simulink model "wb_spectrometer_16"  (R2012b)
(part 2 of 131)

  posedge1 : Subsystem  AncestorBlock=casper_library_misc/edge_detect  mask(edge_detect){edge=Rising, polarity=Active High, x_in=[0 0.08 0.08 0.16 0.16 0.24 0.24 0.32 0.32 0.4], y_in=[-1 -1  1  1  1  1  1  1  1  1], x_out=[0.6 0.68 0.68 0.76 0.76 0.84 0.84 0.92 0.92 1], y_out=[-1 -1  1  1 -1 -1 -1 -1 -1 -1]}
      mask prompts: edge "Edge Type"; polarity "Output Polarity"; x_in "Input X Positions"; y_in "Input Y Positions"; x_out "Output X Positions"; y_out "Output Y Positions"
      mask help: Output is active for one-cycle after each edge of the specified type (i.e. rising, falling or both).
      mask init: same as wb_spectrometer_16/posedge
      settings: AttributesFormatString=|
      | rising edges
      | active high
      mask Help: Output is active for one-cycle after each edge of the specified type (i.e. rising, falling, or both).  Latency is zero.
      mask TypeOptions edge: Rising | Falling | Both
      mask TypeOptions polarity: Active High | Active Low
      mask Display:
      | plot(x_in_num,0.5+y_in_num*0.2);
      | plot(x_out_num,0.5+y_out_num*0.2);
  posedge10 : Subsystem  AncestorBlock=casper_library_misc/edge_detect  mask(edge_detect){edge=Rising, polarity=Active High, x_in=[0 0.08 0.08 0.16 0.16 0.24 0.24 0.32 0.32 0.4], y_in=[-1 -1  1  1  1  1  1  1  1  1], x_out=[0.6 0.68 0.68 0.76 0.76 0.84 0.84 0.92 0.92 1], y_out=[-1 -1  1  1 -1 -1 -1 -1 -1 -1]}
      mask prompts: edge "Edge Type"; polarity "Output Polarity"; x_in "Input X Positions"; y_in "Input Y Positions"; x_out "Output X Positions"; y_out "Output Y Positions"
      mask help: Output is active for one-cycle after each edge of the specified type (i.e. rising, falling or both).
      mask init: same as wb_spectrometer_16/posedge
      settings: AttributesFormatString=|
      | rising edges
      | active high
      mask Help: Output is active for one-cycle after each edge of the specified type (i.e. rising, falling, or both).  Latency is zero.
      mask TypeOptions edge: Rising | Falling | Both
      mask TypeOptions polarity: Active High | Active Low
      mask Display:
      | plot(x_in_num,0.5+y_in_num*0.2);
      | plot(x_out_num,0.5+y_out_num*0.2);
  posedge11 : Subsystem  AncestorBlock=casper_library_misc/edge_detect  mask(edge_detect){edge=Rising, polarity=Active High, x_in=[0 0.08 0.08 0.16 0.16 0.24 0.24 0.32 0.32 0.4], y_in=[-1 -1  1  1  1  1  1  1  1  1], x_out=[0.6 0.68 0.68 0.76 0.76 0.84 0.84 0.92 0.92 1], y_out=[-1 -1  1  1 -1 -1 -1 -1 -1 -1]}
      mask prompts: edge "Edge Type"; polarity "Output Polarity"; x_in "Input X Positions"; y_in "Input Y Positions"; x_out "Output X Positions"; y_out "Output Y Positions"
      mask help: Output is active for one-cycle after each edge of the specified type (i.e. rising, falling or both).
      mask init: same as wb_spectrometer_16/posedge
      settings: AttributesFormatString=|
      | rising edges
      | active high
      mask Help: Output is active for one-cycle after each edge of the specified type (i.e. rising, falling, or both).  Latency is zero.
      mask TypeOptions edge: Rising | Falling | Both
      mask TypeOptions polarity: Active High | Active Low
      mask Display:
      | plot(x_in_num,0.5+y_in_num*0.2);
      | plot(x_out_num,0.5+y_out_num*0.2);
  posedge12 : Subsystem  AncestorBlock=casper_library_misc/edge_detect  mask(edge_detect){edge=Rising, polarity=Active High, x_in=[0 0.08 0.08 0.16 0.16 0.24 0.24 0.32 0.32 0.4], y_in=[-1 -1  1  1  1  1  1  1  1  1], x_out=[0.6 0.68 0.68 0.76 0.76 0.84 0.84 0.92 0.92 1], y_out=[-1 -1  1  1 -1 -1 -1 -1 -1 -1]}
      mask prompts: edge "Edge Type"; polarity "Output Polarity"; x_in "Input X Positions"; y_in "Input Y Positions"; x_out "Output X Positions"; y_out "Output Y Positions"
      mask help: Output is active for one-cycle after each edge of the specified type (i.e. rising, falling or both).
      mask init: same as wb_spectrometer_16/posedge
      settings: AttributesFormatString=|
      | rising edges
      | active high
      mask Help: Output is active for one-cycle after each edge of the specified type (i.e. rising, falling, or both).  Latency is zero.
      mask TypeOptions edge: Rising | Falling | Both
      mask TypeOptions polarity: Active High | Active Low
      mask Display:
      | plot(x_in_num,0.5+y_in_num*0.2);
      | plot(x_out_num,0.5+y_out_num*0.2);
  posedge13 : Subsystem  AncestorBlock=casper_library_misc/edge_detect  mask(edge_detect){edge=Rising, polarity=Active High, x_in=[0 0.08 0.08 0.16 0.16 0.24 0.24 0.32 0.32 0.4], y_in=[-1 -1  1  1  1  1  1  1  1  1], x_out=[0.6 0.68 0.68 0.76 0.76 0.84 0.84 0.92 0.92 1], y_out=[-1 -1  1  1 -1 -1 -1 -1 -1 -1]}
      mask prompts: edge "Edge Type"; polarity "Output Polarity"; x_in "Input X Positions"; y_in "Input Y Positions"; x_out "Output X Positions"; y_out "Output Y Positions"
      mask help: Output is active for one-cycle after each edge of the specified type (i.e. rising, falling or both).
      mask init: same as wb_spectrometer_16/posedge
      settings: AttributesFormatString=|
      | rising edges
      | active high
      mask Help: Output is active for one-cycle after each edge of the specified type (i.e. rising, falling, or both).  Latency is zero.
      mask TypeOptions edge: Rising | Falling | Both
      mask TypeOptions polarity: Active High | Active Low
      mask Display:
      | plot(x_in_num,0.5+y_in_num*0.2);
      | plot(x_out_num,0.5+y_out_num*0.2);
  posedge14 : Subsystem  AncestorBlock=casper_library_misc/edge_detect  mask(edge_detect){edge=Rising, polarity=Active High, x_in=[0 0.08 0.08 0.16 0.16 0.24 0.24 0.32 0.32 0.4], y_in=[-1 -1  1  1  1  1  1  1  1  1], x_out=[0.6 0.68 0.68 0.76 0.76 0.84 0.84 0.92 0.92 1], y_out=[-1 -1  1  1 -1 -1 -1 -1 -1 -1]}
      mask prompts: edge "Edge Type"; polarity "Output Polarity"; x_in "Input X Positions"; y_in "Input Y Positions"; x_out "Output X Positions"; y_out "Output Y Positions"
      mask help: Output is active for one-cycle after each edge of the specified type (i.e. rising, falling or both).
      mask init: same as wb_spectrometer_16/posedge
      settings: AttributesFormatString=|
      | rising edges
      | active high
      mask Help: Output is active for one-cycle after each edge of the specified type (i.e. rising, falling, or both).  Latency is zero.
      mask TypeOptions edge: Rising | Falling | Both
      mask TypeOptions polarity: Active High | Active Low
      mask Display:
      | plot(x_in_num,0.5+y_in_num*0.2);
      | plot(x_out_num,0.5+y_out_num*0.2);
  posedge15 : Subsystem  AncestorBlock=casper_library_misc/edge_detect  mask(edge_detect){edge=Rising, polarity=Active High, x_in=[0 0.08 0.08 0.16 0.16 0.24 0.24 0.32 0.32 0.4], y_in=[-1 -1  1  1  1  1  1  1  1  1], x_out=[0.6 0.68 0.68 0.76 0.76 0.84 0.84 0.92 0.92 1], y_out=[-1 -1  1  1 -1 -1 -1 -1 -1 -1]}
      mask prompts: edge "Edge Type"; polarity "Output Polarity"; x_in "Input X Positions"; y_in "Input Y Positions"; x_out "Output X Positions"; y_out "Output Y Positions"
      mask help: Output is active for one-cycle after each edge of the specified type (i.e. rising, falling or both).
      mask init: same as wb_spectrometer_16/posedge
      settings: AttributesFormatString=|
      | rising edges
      | active high
      mask Help: Output is active for one-cycle after each edge of the specified type (i.e. rising, falling, or both).  Latency is zero.
      mask TypeOptions edge: Rising | Falling | Both
      mask TypeOptions polarity: Active High | Active Low
      mask Display:
      | plot(x_in_num,0.5+y_in_num*0.2);
      | plot(x_out_num,0.5+y_out_num*0.2);
  posedge16 : Subsystem  AncestorBlock=casper_library_misc/edge_detect  mask(edge_detect){edge=Rising, polarity=Active High, x_in=[0 0.08 0.08 0.16 0.16 0.24 0.24 0.32 0.32 0.4], y_in=[-1 -1  1  1  1  1  1  1  1  1], x_out=[0.6 0.68 0.68 0.76 0.76 0.84 0.84 0.92 0.92 1], y_out=[-1 -1  1  1 -1 -1 -1 -1 -1 -1]}
      mask prompts: edge "Edge Type"; polarity "Output Polarity"; x_in "Input X Positions"; y_in "Input Y Positions"; x_out "Output X Positions"; y_out "Output Y Positions"
      mask help: Output is active for one-cycle after each edge of the specified type (i.e. rising, falling or both).
      mask init: same as wb_spectrometer_16/posedge
      settings: AttributesFormatString=|
      | rising edges
      | active high
      mask Help: Output is active for one-cycle after each edge of the specified type (i.e. rising, falling, or both).  Latency is zero.
      mask TypeOptions edge: Rising | Falling | Both
      mask TypeOptions polarity: Active High | Active Low
      mask Display:
      | plot(x_in_num,0.5+y_in_num*0.2);
      | plot(x_out_num,0.5+y_out_num*0.2);
  posedge17 : Subsystem  AncestorBlock=casper_library_misc/edge_detect  mask(edge_detect){edge=Falling, polarity=Active High, x_in=[0 0.08 0.08 0.16 0.16 0.24 0.24 0.32 0.32 0.4], y_in=[-1 -1  1  1  1  1  1  1  1  1], x_out=[0.6 0.68 0.68 0.76 0.76 0.84 0.84 0.92 0.92 1], y_out=[-1 -1  1  1 -1 -1 -1 -1 -1 -1]}
      mask prompts: edge "Edge Type"; polarity "Output Polarity"; x_in "Input X Positions"; y_in "Input Y Positions"; x_out "Output X Positions"; y_out "Output Y Positions"
      mask help: Output is active for one-cycle after each edge of the specified type (i.e. rising, falling or both).
      mask init: same as wb_spectrometer_16/posedge
      settings: AttributesFormatString=|
      | falling edges
      | active high
      mask Help: Output is active for one-cycle after each edge of the specified type (i.e. rising, falling, or both).  Latency is zero.
      mask TypeOptions edge: Rising | Falling | Both
      mask TypeOptions polarity: Active High | Active Low
      mask Display:
      | plot(x_in_num,0.5+y_in_num*0.2);
      | plot(x_out_num,0.5+y_out_num*0.2);
  posedge18 : Subsystem  AncestorBlock=casper_library_misc/edge_detect  mask(edge_detect){edge=Rising, polarity=Active High, x_in=[0 0.08 0.08 0.16 0.16 0.24 0.24 0.32 0.32 0.4], y_in=[-1 -1  1  1  1  1  1  1  1  1], x_out=[0.6 0.68 0.68 0.76 0.76 0.84 0.84 0.92 0.92 1], y_out=[-1 -1  1  1 -1 -1 -1 -1 -1 -1]}
      mask prompts: edge "Edge Type"; polarity "Output Polarity"; x_in "Input X Positions"; y_in "Input Y Positions"; x_out "Output X Positions"; y_out "Output Y Positions"
      mask help: Output is active for one-cycle after each edge of the specified type (i.e. rising, falling or both).
      mask init: same as wb_spectrometer_16/posedge
      settings: AttributesFormatString=|
      | rising edges
      | active high
      mask Help: Output is active for one-cycle after each edge of the specified type (i.e. rising, falling, or both).  Latency is zero.
      mask TypeOptions edge: Rising | Falling | Both
      mask TypeOptions polarity: Active High | Active Low
      mask Display:
      | plot(x_in_num,0.5+y_in_num*0.2);
      | plot(x_out_num,0.5+y_out_num*0.2);
  posedge19 : Subsystem  AncestorBlock=casper_library_misc/edge_detect  mask(edge_detect){edge=Rising, polarity=Active High, x_in=[0 0.08 0.08 0.16 0.16 0.24 0.24 0.32 0.32 0.4], y_in=[-1 -1  1  1  1  1  1  1  1  1], x_out=[0.6 0.68 0.68 0.76 0.76 0.84 0.84 0.92 0.92 1], y_out=[-1 -1  1  1 -1 -1 -1 -1 -1 -1]}
      mask prompts: edge "Edge Type"; polarity "Output Polarity"; x_in "Input X Positions"; y_in "Input Y Positions"; x_out "Output X Positions"; y_out "Output Y Positions"
      mask help: Output is active for one-cycle after each edge of the specified type (i.e. rising, falling or both).
      mask init: same as wb_spectrometer_16/posedge
      settings: AttributesFormatString=|
      | rising edges
      | active high
      mask Help: Output is active for one-cycle after each edge of the specified type (i.e. rising, falling, or both).  Latency is zero.
      mask TypeOptions edge: Rising | Falling | Both
      mask TypeOptions polarity: Active High | Active Low
      mask Display:
      | plot(x_in_num,0.5+y_in_num*0.2);
      | plot(x_out_num,0.5+y_out_num*0.2);
  posedge2 : Subsystem  AncestorBlock=casper_library_misc/edge_detect  mask(edge_detect){edge=Rising, polarity=Active High, x_in=[0 0.08 0.08 0.16 0.16 0.24 0.24 0.32 0.32 0.4], y_in=[-1 -1  1  1  1  1  1  1  1  1], x_out=[0.6 0.68 0.68 0.76 0.76 0.84 0.84 0.92 0.92 1], y_out=[-1 -1  1  1 -1 -1 -1 -1 -1 -1]}
      mask prompts: edge "Edge Type"; polarity "Output Polarity"; x_in "Input X Positions"; y_in "Input Y Positions"; x_out "Output X Positions"; y_out "Output Y Positions"
      mask help: Output is active for one-cycle after each edge of the specified type (i.e. rising, falling or both).
      mask init: same as wb_spectrometer_16/posedge
      settings: AttributesFormatString=|
      | rising edges
      | active high
      mask Help: Output is active for one-cycle after each edge of the specified type (i.e. rising, falling, or both).  Latency is zero.
      mask TypeOptions edge: Rising | Falling | Both
      mask TypeOptions polarity: Active High | Active Low
      mask Display:
      | plot(x_in_num,0.5+y_in_num*0.2);
      | plot(x_out_num,0.5+y_out_num*0.2);
  posedge3 : Subsystem  AncestorBlock=casper_library_misc/edge_detect  mask(edge_detect){edge=Rising, polarity=Active High, x_in=[0 0.08 0.08 0.16 0.16 0.24 0.24 0.32 0.32 0.4], y_in=[-1 -1  1  1  1  1  1  1  1  1], x_out=[0.6 0.68 0.68 0.76 0.76 0.84 0.84 0.92 0.92 1], y_out=[-1 -1  1  1 -1 -1 -1 -1 -1 -1]}
      mask prompts: edge "Edge Type"; polarity "Output Polarity"; x_in "Input X Positions"; y_in "Input Y Positions"; x_out "Output X Positions"; y_out "Output Y Positions"
      mask help: Output is active for one-cycle after each edge of the specified type (i.e. rising, falling or both).
      mask init: same as wb_spectrometer_16/posedge
      settings: AttributesFormatString=|
      | rising edges
      | active high
      mask Help: Output is active for one-cycle after each edge of the specified type (i.e. rising, falling, or both).  Latency is zero.
      mask TypeOptions edge: Rising | Falling | Both
      mask TypeOptions polarity: Active High | Active Low
      mask Display:
      | plot(x_in_num,0.5+y_in_num*0.2);
      | plot(x_out_num,0.5+y_out_num*0.2);
  posedge4 : Subsystem  AncestorBlock=casper_library_misc/edge_detect  mask(edge_detect){edge=Rising, polarity=Active High, x_in=[0 0.08 0.08 0.16 0.16 0.24 0.24 0.32 0.32 0.4], y_in=[-1 -1  1  1  1  1  1  1  1  1], x_out=[0.6 0.68 0.68 0.76 0.76 0.84 0.84 0.92 0.92 1], y_out=[-1 -1  1  1 -1 -1 -1 -1 -1 -1]}
      mask prompts: edge "Edge Type"; polarity "Output Polarity"; x_in "Input X Positions"; y_in "Input Y Positions"; x_out "Output X Positions"; y_out "Output Y Positions"
      mask help: Output is active for one-cycle after each edge of the specified type (i.e. rising, falling or both).
      mask init: same as wb_spectrometer_16/posedge
      settings: AttributesFormatString=|
      | rising edges
      | active high
      mask Help: Output is active for one-cycle after each edge of the specified type (i.e. rising, falling, or both).  Latency is zero.
      mask TypeOptions edge: Rising | Falling | Both
      mask TypeOptions polarity: Active High | Active Low
      mask Display:
      | plot(x_in_num,0.5+y_in_num*0.2);
      | plot(x_out_num,0.5+y_out_num*0.2);
  posedge5 : Subsystem  AncestorBlock=casper_library_misc/edge_detect  mask(edge_detect){edge=Rising, polarity=Active High, x_in=[0 0.08 0.08 0.16 0.16 0.24 0.24 0.32 0.32 0.4], y_in=[-1 -1  1  1  1  1  1  1  1  1], x_out=[0.6 0.68 0.68 0.76 0.76 0.84 0.84 0.92 0.92 1], y_out=[-1 -1  1  1 -1 -1 -1 -1 -1 -1]}
      mask prompts: edge "Edge Type"; polarity "Output Polarity"; x_in "Input X Positions"; y_in "Input Y Positions"; x_out "Output X Positions"; y_out "Output Y Positions"
      mask help: Output is active for one-cycle after each edge of the specified type (i.e. rising, falling or both).
      mask init: same as wb_spectrometer_16/posedge
      settings: AttributesFormatString=|
      | rising edges
      | active high
      mask Help: Output is active for one-cycle after each edge of the specified type (i.e. rising, falling, or both).  Latency is zero.
      mask TypeOptions edge: Rising | Falling | Both
      mask TypeOptions polarity: Active High | Active Low
      mask Display:
      | plot(x_in_num,0.5+y_in_num*0.2);
      | plot(x_out_num,0.5+y_out_num*0.2);
  posedge6 : Subsystem  AncestorBlock=casper_library_misc/edge_detect  mask(edge_detect){edge=Rising, polarity=Active High, x_in=[0 0.08 0.08 0.16 0.16 0.24 0.24 0.32 0.32 0.4], y_in=[-1 -1  1  1  1  1  1  1  1  1], x_out=[0.6 0.68 0.68 0.76 0.76 0.84 0.84 0.92 0.92 1], y_out=[-1 -1  1  1 -1 -1 -1 -1 -1 -1]}
      mask prompts: edge "Edge Type"; polarity "Output Polarity"; x_in "Input X Positions"; y_in "Input Y Positions"; x_out "Output X Positions"; y_out "Output Y Positions"
      mask help: Output is active for one-cycle after each edge of the specified type (i.e. rising, falling or both).
      mask init: same as wb_spectrometer_16/posedge
      settings: AttributesFormatString=|
      | rising edges
      | active high
      mask Help: Output is active for one-cycle after each edge of the specified type (i.e. rising, falling, or both).  Latency is zero.
      mask TypeOptions edge: Rising | Falling | Both
      mask TypeOptions polarity: Active High | Active Low
      mask Display:
      | plot(x_in_num,0.5+y_in_num*0.2);
      | plot(x_out_num,0.5+y_out_num*0.2);
  posedge8 : Subsystem  AncestorBlock=casper_library_misc/edge_detect  mask(edge_detect){edge=Rising, polarity=Active High, x_in=[0 0.08 0.08 0.16 0.16 0.24 0.24 0.32 0.32 0.4], y_in=[-1 -1  1  1  1  1  1  1  1  1], x_out=[0.6 0.68 0.68 0.76 0.76 0.84 0.84 0.92 0.92 1], y_out=[-1 -1  1  1 -1 -1 -1 -1 -1 -1]}
      mask prompts: edge "Edge Type"; polarity "Output Polarity"; x_in "Input X Positions"; y_in "Input Y Positions"; x_out "Output X Positions"; y_out "Output Y Positions"
      mask help: Output is active for one-cycle after each edge of the specified type (i.e. rising, falling or both).
      mask init: same as wb_spectrometer_16/posedge
      settings: AttributesFormatString=|
      | rising edges
      | active high
      mask Help: Output is active for one-cycle after each edge of the specified type (i.e. rising, falling, or both).  Latency is zero.
      mask TypeOptions edge: Rising | Falling | Both
      mask TypeOptions polarity: Active High | Active Low
      mask Display:
      | plot(x_in_num,0.5+y_in_num*0.2);
      | plot(x_out_num,0.5+y_out_num*0.2);
  posedge9 : Subsystem  AncestorBlock=casper_library_misc/edge_detect  mask(edge_detect){edge=Rising, polarity=Active High, x_in=[0 0.08 0.08 0.16 0.16 0.24 0.24 0.32 0.32 0.4], y_in=[-1 -1  1  1  1  1  1  1  1  1], x_out=[0.6 0.68 0.68 0.76 0.76 0.84 0.84 0.92 0.92 1], y_out=[-1 -1  1  1 -1 -1 -1 -1 -1 -1]}
      mask prompts: edge "Edge Type"; polarity "Output Polarity"; x_in "Input X Positions"; y_in "Input Y Positions"; x_out "Output X Positions"; y_out "Output Y Positions"
      mask help: Output is active for one-cycle after each edge of the specified type (i.e. rising, falling or both).
      mask init: same as wb_spectrometer_16/posedge
      settings: AttributesFormatString=|
      | rising edges
      | active high
      mask Help: Output is active for one-cycle after each edge of the specified type (i.e. rising, falling, or both).  Latency is zero.
      mask TypeOptions edge: Rising | Falling | Both
      mask TypeOptions polarity: Active High | Active Low
      mask Display:
      | plot(x_in_num,0.5+y_in_num*0.2);
      | plot(x_out_num,0.5+y_out_num*0.2);
  pps_ : xbsIndex_r4/Gateway Out  inherit_from_input=off  hdl_port=on  timing_constraint=None  locs_specified=off  LOCs={}  UseAsDAC=off  DACChannel='1'  block_type=gatewayout
  pps_cnt : Subsystem  Tag=xps:sw_reg  AncestorBlock=xps_library/software register  mask(swreg){mode=one value, io_dir=To Processor, io_delay=0, sample_period=1, names=reg, bitwidths=32, arith_types=0, bin_pts=0, sim_port=on, show_format=off}
      mask prompts: io_dir "I/O direction"; io_delay "I/O delay"; sample_period "Sample period"; names "Name:"; bitwidths "Bitwidth:"; arith_types "Type (ufix=0, fix=1, bool=2):"; bin_pts "Binary pt:"; sim_port "Provide sim input/output?"; show_format "Print format string?"
      mask init:
      | swreg_init(gcb)
      settings: AttributesFormatString=1output
      mask TypeOptions mode: one value | fields of equal size | fields of arbitrary size
      mask Callback mode: swreg_cb(gcb);
      mask TypeOptions io_dir: To Processor | From Processor
      mask Callback io_dir:
      | mask_enables = get_param(gcb, 'MaskEnables');
      | mask_names = get_param(gcb, 'MaskNames');
      | if strcmp(get_param(gcb, 'io_dir'), 'To Processor'),
      |     mask_enables{ismember(mask_names, 'sample_period')} = 'off';
      | else
      |     mask_enables{ismember(mask_names, 'sample_period')} = 'on';
      | end
      | set_param(gcb, 'MaskEnables', mask_enables);
      mask Callback bitwidths: swreg_maskcheck(gcb);
      mask Callback arith_types: [numios, ~, ~, ~, current_types] = swreg_maskcheck(gcb);
      mask Callback bin_pts: swreg_maskcheck(gcb);
  queue_empty : Subsystem  Tag=xps:sw_reg  AncestorBlock=xps_library/software register  mask(swreg){mode=one value, io_dir=To Processor, io_delay=0, sample_period=1, names=reg, bitwidths=1, arith_types=2, bin_pts=0, sim_port=on, show_format=off}
      mask prompts: io_dir "I/O direction"; io_delay "I/O delay"; sample_period "Sample period"; names "Name:"; bitwidths "Bitwidth:"; arith_types "Type (ufix=0, fix=1, bool=2):"; bin_pts "Binary pt:"; sim_port "Provide sim input/output?"; show_format "Print format string?"
      mask init:
      | swreg_init(gcb)
      settings: AttributesFormatString=1output
      mask TypeOptions mode: one value | fields of equal size | fields of arbitrary size
      mask Callback mode: swreg_cb(gcb);
      mask TypeOptions io_dir: To Processor | From Processor
      mask Callback io_dir:
      | mask_enables = get_param(gcb, 'MaskEnables');
      | mask_names = get_param(gcb, 'MaskNames');
      | if strcmp(get_param(gcb, 'io_dir'), 'To Processor'),
      |     mask_enables{ismember(mask_names, 'sample_period')} = 'off';
      | else
      |     mask_enables{ismember(mask_names, 'sample_period')} = 'on';
      | end
      | set_param(gcb, 'MaskEnables', mask_enables);
      mask Callback bitwidths: swreg_maskcheck(gcb);
      mask Callback arith_types: [numios, ~, ~, ~, current_types] = swreg_maskcheck(gcb);
      mask Callback bin_pts: swreg_maskcheck(gcb);
  queue_perc_full : Subsystem  Tag=xps:sw_reg  AncestorBlock=xps_library/software register  mask(swreg){mode=one value, io_dir=To Processor, io_delay=0, sample_period=1, names=reg, bitwidths=8, arith_types=0, bin_pts=8, sim_port=on, show_format=off}
      mask prompts: io_dir "I/O direction"; io_delay "I/O delay"; sample_period "Sample period"; names "Name:"; bitwidths "Bitwidth:"; arith_types "Type (ufix=0, fix=1, bool=2):"; bin_pts "Binary pt:"; sim_port "Provide sim input/output?"; show_format "Print format string?"
      mask init:
      | swreg_init(gcb)
      settings: AttributesFormatString=1output
      mask TypeOptions mode: one value | fields of equal size | fields of arbitrary size
      mask Callback mode: swreg_cb(gcb);
      mask TypeOptions io_dir: To Processor | From Processor
      mask Callback io_dir:
      | mask_enables = get_param(gcb, 'MaskEnables');
      | mask_names = get_param(gcb, 'MaskNames');
      | if strcmp(get_param(gcb, 'io_dir'), 'To Processor'),
      |     mask_enables{ismember(mask_names, 'sample_period')} = 'off';
      | else
      |     mask_enables{ismember(mask_names, 'sample_period')} = 'on';
      | end
      | set_param(gcb, 'MaskEnables', mask_enables);
      mask Callback bitwidths: swreg_maskcheck(gcb);
      mask Callback arith_types: [numios, ~, ~, ~, current_types] = swreg_maskcheck(gcb);
      mask Callback bin_pts: swreg_maskcheck(gcb);
  roach_gpio_a_enable_not : xps_library/gpio  Tag=xps:gpio  io_group=ROACH:gpioa_oe_n  io_dir=out  arith_type=Boolean  bitwidth=1  bin_pt=0  bit_index=0  sample_period=1  use_single_ended=off  use_ddr=off  reg_iob=off  reg_clk_phase=0  termination=None
      link override convert: arith_type=Boolean  n_bits=1  bin_pt=0
  roach_gpio_b_enable_not : xps_library/gpio  Tag=xps:gpio  io_group=ROACH:gpiob_oe_n  io_dir=out  arith_type=Boolean  bitwidth=1  bin_pt=0  bit_index=0  sample_period=1  use_single_ended=off  use_ddr=off  reg_iob=off  reg_clk_phase=0  termination=None
      link override convert: arith_type=Boolean  n_bits=1  bin_pt=0
  roach_led0 : xps_library/gpio  Tag=xps:gpio  io_group=ROACH:gpiob  io_dir=out  arith_type=Boolean  bitwidth=1  bin_pt=0  bit_index=0  sample_period=1  use_single_ended=off  use_ddr=off  reg_iob=off  reg_clk_phase=0  termination=None
      link override convert: arith_type=Boolean  n_bits=1  bin_pt=0
  roach_led1 : xps_library/gpio  Tag=xps:gpio  io_group=ROACH:gpiob  io_dir=out  arith_type=Boolean  bitwidth=1  bin_pt=0  bit_index=1  sample_period=1  use_single_ended=off  use_ddr=off  reg_iob=off  reg_clk_phase=0  termination=None
      link override convert: arith_type=Boolean  n_bits=1  bin_pt=0
  roach_led2 : xps_library/gpio  Tag=xps:gpio  io_group=ROACH:gpiob  io_dir=out  arith_type=Boolean  bitwidth=1  bin_pt=0  bit_index=2  sample_period=1  use_single_ended=off  use_ddr=off  reg_iob=off  reg_clk_phase=0  termination=None
      link override convert: arith_type=Boolean  n_bits=1  bin_pt=0
  roach_led3 : xps_library/gpio  Tag=xps:gpio  io_group=ROACH:gpiob  io_dir=out  arith_type=Boolean  bitwidth=1  bin_pt=0  bit_index=3  sample_period=1  use_single_ended=off  use_ddr=off  reg_iob=off  reg_clk_phase=0  termination=None
      link override convert: arith_type=Boolean  n_bits=1  bin_pt=0
  roach_led4 : xps_library/gpio  Tag=xps:gpio  io_group=ROACH:gpiob  io_dir=out  arith_type=Boolean  bitwidth=1  bin_pt=0  bit_index=4  sample_period=1  use_single_ended=off  use_ddr=off  reg_iob=off  reg_clk_phase=0  termination=None
      link override convert: arith_type=Boolean  n_bits=1  bin_pt=0
  roach_led5 : xps_library/gpio  Tag=xps:gpio  io_group=ROACH:gpiob  io_dir=out  arith_type=Boolean  bitwidth=1  bin_pt=0  bit_index=5  sample_period=1  use_single_ended=off  use_ddr=off  reg_iob=off  reg_clk_phase=0  termination=None
      link override convert: arith_type=Boolean  n_bits=1  bin_pt=0
  roach_led6 : xps_library/gpio  Tag=xps:gpio  io_group=ROACH:gpiob  io_dir=out  arith_type=Boolean  bitwidth=1  bin_pt=0  bit_index=6  sample_period=1  use_single_ended=off  use_ddr=off  reg_iob=off  reg_clk_phase=0  termination=None
      link override convert: arith_type=Boolean  n_bits=1  bin_pt=0
  roach_led7 : xps_library/gpio  Tag=xps:gpio  io_group=ROACH:gpiob  io_dir=out  arith_type=Boolean  bitwidth=1  bin_pt=0  bit_index=7  sample_period=1  use_single_ended=off  use_ddr=off  reg_iob=off  reg_clk_phase=0  termination=None
      link override convert: arith_type=Boolean  n_bits=1  bin_pt=0
  roach_sma_j10 : xps_library/gpio  Tag=xps:gpio  io_group=ROACH:gpioa  io_dir=out  arith_type=Boolean  bitwidth=1  bin_pt=0  bit_index=4  sample_period=1  use_single_ended=off  use_ddr=off  reg_iob=off  reg_clk_phase=0  termination=None
      link override convert: arith_type=Boolean  n_bits=1  bin_pt=0
  rtc_ : xbsIndex_r4/Gateway Out  inherit_from_input=off  hdl_port=on  timing_constraint=None  locs_specified=off  LOCs={}  UseAsDAC=off  DACChannel='1'  block_type=gatewayout
  sampling_frequency_mhz : Subsystem  Tag=xps:sw_reg  AncestorBlock=xps_library/software register  mask(swreg){mode=one value, io_dir=To Processor, io_delay=0, sample_period=1, names=reg, bitwidths=32, arith_types=0, bin_pts=0, sim_port=on, show_format=off}
      mask prompts: io_dir "I/O direction"; io_delay "I/O delay"; sample_period "Sample period"; names "Name:"; bitwidths "Bitwidth:"; arith_types "Type (ufix=0, fix=1, bool=2):"; bin_pts "Binary pt:"; sim_port "Provide sim input/output?"; show_format "Print format string?"
      mask init:
      | swreg_init(gcb)
      settings: AttributesFormatString=1output
      mask TypeOptions mode: one value | fields of equal size | fields of arbitrary size
      mask Callback mode: swreg_cb(gcb);
      mask TypeOptions io_dir: To Processor | From Processor
      mask Callback io_dir:
      | mask_enables = get_param(gcb, 'MaskEnables');
      | mask_names = get_param(gcb, 'MaskNames');
      | if strcmp(get_param(gcb, 'io_dir'), 'To Processor'),
      |     mask_enables{ismember(mask_names, 'sample_period')} = 'off';
      | else
      |     mask_enables{ismember(mask_names, 'sample_period')} = 'on';
      | end
      | set_param(gcb, 'MaskEnables', mask_enables);
      mask Callback bitwidths: swreg_maskcheck(gcb);
      mask Callback arith_types: [numios, ~, ~, ~, current_types] = swreg_maskcheck(gcb);
      mask Callback bin_pts: swreg_maskcheck(gcb);
  simple_bram_vacc_i_even : Subsystem  AncestorBlock=casper_library_accumulators/simple_bram_vacc  mask(simple_bram_vacc){vec_len=512, arith_type=Signed, n_bits=32, bin_pt=0}
      mask prompts: vec_len "Vector length:"; arith_type "Output type:"; n_bits "Bit width (output):"; bin_pt "Binary point (output):"
      mask help: This simple vector accumulator is based on a shift register. It outputs its previous accumulated vector after a new_acc pulse is received.
      mask init:
      | simple_bram_vacc_init(gcb, ...
      |     'vec_len', vec_len, ...
      |     'arith_type', arith_type, ...
      |     'n_bits', n_bits, ...
      |     'bin_pt', bin_pt);
      mask TypeOptions arith_type: Signed | Unsigned
  simple_bram_vacc_i_odd : Subsystem  AncestorBlock=casper_library_accumulators/simple_bram_vacc  mask(simple_bram_vacc){vec_len=512, arith_type=Signed, n_bits=32, bin_pt=0}
      mask prompts: vec_len "Vector length:"; arith_type "Output type:"; n_bits "Bit width (output):"; bin_pt "Binary point (output):"
      mask help: This simple vector accumulator is based on a shift register. It outputs its previous accumulated vector after a new_acc pulse is received.
      mask init:
      | simple_bram_vacc_init(gcb, ...
      |     'vec_len', vec_len, ...
      |     'arith_type', arith_type, ...
      |     'n_bits', n_bits, ...
      |     'bin_pt', bin_pt);
      mask TypeOptions arith_type: Signed | Unsigned
  simple_bram_vacc_q_even : Subsystem  AncestorBlock=casper_library_accumulators/simple_bram_vacc  mask(simple_bram_vacc){vec_len=512, arith_type=Signed, n_bits=32, bin_pt=0}
      mask prompts: vec_len "Vector length:"; arith_type "Output type:"; n_bits "Bit width (output):"; bin_pt "Binary point (output):"
      mask help: This simple vector accumulator is based on a shift register. It outputs its previous accumulated vector after a new_acc pulse is received.
      mask init:
      | simple_bram_vacc_init(gcb, ...
      |     'vec_len', vec_len, ...
      |     'arith_type', arith_type, ...
      |     'n_bits', n_bits, ...
      |     'bin_pt', bin_pt);
      mask TypeOptions arith_type: Signed | Unsigned
  simple_bram_vacc_q_odd : Subsystem  AncestorBlock=casper_library_accumulators/simple_bram_vacc  mask(simple_bram_vacc){vec_len=512, arith_type=Signed, n_bits=32, bin_pt=0}
      mask prompts: vec_len "Vector length:"; arith_type "Output type:"; n_bits "Bit width (output):"; bin_pt "Binary point (output):"
      mask help: This simple vector accumulator is based on a shift register. It outputs its previous accumulated vector after a new_acc pulse is received.
      mask init:
      | simple_bram_vacc_init(gcb, ...
      |     'vec_len', vec_len, ...
      |     'arith_type', arith_type, ...
      |     'n_bits', n_bits, ...
      |     'bin_pt', bin_pt);
      mask TypeOptions arith_type: Signed | Unsigned
  simple_bram_vacc_u_even : Subsystem  AncestorBlock=casper_library_accumulators/simple_bram_vacc  mask(simple_bram_vacc){vec_len=512, arith_type=Signed, n_bits=32, bin_pt=0}
      mask prompts: vec_len "Vector length:"; arith_type "Output type:"; n_bits "Bit width (output):"; bin_pt "Binary point (output):"
      mask help: This simple vector accumulator is based on a shift register. It outputs its previous accumulated vector after a new_acc pulse is received.
      mask init:
      | simple_bram_vacc_init(gcb, ...
      |     'vec_len', vec_len, ...
      |     'arith_type', arith_type, ...
      |     'n_bits', n_bits, ...
      |     'bin_pt', bin_pt);
      mask TypeOptions arith_type: Signed | Unsigned
  simple_bram_vacc_u_odd : Subsystem  AncestorBlock=casper_library_accumulators/simple_bram_vacc  mask(simple_bram_vacc){vec_len=512, arith_type=Signed, n_bits=32, bin_pt=0}
      mask prompts: vec_len "Vector length:"; arith_type "Output type:"; n_bits "Bit width (output):"; bin_pt "Binary point (output):"
      mask help: This simple vector accumulator is based on a shift register. It outputs its previous accumulated vector after a new_acc pulse is received.
      mask init:
      | simple_bram_vacc_init(gcb, ...
      |     'vec_len', vec_len, ...
      |     'arith_type', arith_type, ...
      |     'n_bits', n_bits, ...
      |     'bin_pt', bin_pt);
      mask TypeOptions arith_type: Signed | Unsigned
  simple_bram_vacc_v_even : Subsystem  AncestorBlock=casper_library_accumulators/simple_bram_vacc  mask(simple_bram_vacc){vec_len=512, arith_type=Signed, n_bits=32, bin_pt=0}
      mask prompts: vec_len "Vector length:"; arith_type "Output type:"; n_bits "Bit width (output):"; bin_pt "Binary point (output):"
      mask help: This simple vector accumulator is based on a shift register. It outputs its previous accumulated vector after a new_acc pulse is received.
      mask init:
      | simple_bram_vacc_init(gcb, ...
      |     'vec_len', vec_len, ...
      |     'arith_type', arith_type, ...
      |     'n_bits', n_bits, ...
      |     'bin_pt', bin_pt);
      mask TypeOptions arith_type: Signed | Unsigned
  simple_bram_vacc_v_odd : Subsystem  AncestorBlock=casper_library_accumulators/simple_bram_vacc  mask(simple_bram_vacc){vec_len=512, arith_type=Signed, n_bits=32, bin_pt=0}
      mask prompts: vec_len "Vector length:"; arith_type "Output type:"; n_bits "Bit width (output):"; bin_pt "Binary point (output):"
      mask help: This simple vector accumulator is based on a shift register. It outputs its previous accumulated vector after a new_acc pulse is received.
      mask init:
      | simple_bram_vacc_init(gcb, ...
      |     'vec_len', vec_len, ...
      |     'arith_type', arith_type, ...
      |     'n_bits', n_bits, ...
      |     'bin_pt', bin_pt);
      mask TypeOptions arith_type: Signed | Unsigned
  stokes_enable : Subsystem  Tag=xps:sw_reg  AncestorBlock=xps_library/software register  mask(swreg){mode=one value, io_dir=From Processor, io_delay=0, sample_period=1, names=reg, bitwidths=32, arith_types=0, bin_pts=0, sim_port=on, show_format=off}
      mask prompts: io_dir "I/O direction"; io_delay "I/O delay"; sample_period "Sample period"; names "Name:"; bitwidths "Bitwidth:"; arith_types "Type (ufix=0, fix=1, bool=2):"; bin_pts "Binary pt:"; sim_port "Provide sim input/output?"; show_format "Print format string?"
      mask init:
      | swreg_init(gcb)
      settings: AttributesFormatString=1input
      mask TypeOptions mode: one value | fields of equal size | fields of arbitrary size
      mask Callback mode: swreg_cb(gcb);
      mask TypeOptions io_dir: To Processor | From Processor
      mask Callback io_dir:
      | mask_enables = get_param(gcb, 'MaskEnables');
      | mask_names = get_param(gcb, 'MaskNames');
      | if strcmp(get_param(gcb, 'io_dir'), 'To Processor'),
      |     mask_enables{ismember(mask_names, 'sample_period')} = 'off';
      | else
      |     mask_enables{ismember(mask_names, 'sample_period')} = 'on';
      | end
      | set_param(gcb, 'MaskEnables', mask_enables);
      mask Callback bitwidths:
      | swreg_maskcheck(gcb);
      | % blk = gcb;
      | % mode = get_param(blk, 'mode');
      | % current_widths = eval(get_param(blk, 'bitwidths'));
      | % if (strcmp(mode, 'one value') || strcmp(mode, 'fields of equal size')) && (length(current_widths) > 1),
      | %     error('Only one width may be specified for this mode.');
      | % elseif strcmp(mode, 'fields of arbitrary size')
      | %     current_names = textscan(strtrim(strrep(strrep(get_param(blk, 'names'), ']', ''), '[', '')), '%s');
      | %     current_names = current_names{1};
      | %     numios = length(current_names);
      | %     if length(current_widths) ~= numios,
      | %         error('%d field names specified, but %d widths?', numios, length(current_widths));
      | %     end
      | % end
      | % total_width = 0;
      | % for ctr = 1 : length(current_widths),
      | %     total_width = total_width + current_widths(ctr);
      | % end
      | % if total_width > 32,
      | %     error('Total width must be 32 or less, set to %d.', total_width);
      | % end
      mask Callback arith_types:
      | [numios, ~, ~, ~, current_types] = swreg_maskcheck(gcb);
      | % blk = gcb;
      | % mode = get_param(blk, 'mode');
      | % current_types = eval(get_param(blk, 'arith_types'));
      | % numios = length(current_types);
      | % if (strcmp(mode, 'one value') || strcmp(mode, 'fields of equal size')) && (length(current_types) > 1),
      | %     error('Only one type may be specified for this mode.');
      | % elseif strcmp(mode, 'fields of arbitrary size')
      | %     current_names = textscan(strtrim(strrep(strrep(get_param(blk, 'names'), ']', ''), '[', '')), '%s');
      | %     current_names = current_names{1};
      | %     numios = length(current_names);
      | %     if length(current_types) ~= numios,
      | %         error('%d field names specified, but %d types?', numios, length(current_types));
      | %     end
      | % end
      | problem = 0;
      | for ctr = 1 : numios,
      |     t = current_types(ctr);
      |     if (t < 0) || (t > 2),
      |         problem = t;
      |         ctr = numios + 1;
      |     end
      | end
      | if problem ~= 0,
      |     error('Type cannot be %i, must be 0, 1 or 2.', problem);
      | end
      mask Callback bin_pts:
      | swreg_maskcheck(gcb);
      | % blk = gcb;
      | % mode = get_param(blk, 'mode');
      | % current_bins = eval(get_param(blk, 'bin_pts'));
      | % if (strcmp(mode, 'one value') || strcmp(mode, 'fields of equal size')) && (length(current_bins) > 1),
      | %     error('Only one binary pt may be specified for this mode.');
      | % elseif strcmp(mode, 'fields of arbitrary size')
      | %     current_names = textscan(strtrim(strrep(strrep(get_param(blk, 'names'), ']', ''), '[', '')), '%s');
      | %     current_names = current_names{1};
      | %     numios = length(current_names);
      | %     if length(current_bins) ~= numios,
      | %         error('%d field names specified, but %d binary pts?', numios, length(current_bins));
      | %     end
      | % end
  stokes_even : Subsystem
  stokes_odd : Subsystem
  sub_frame_cnt : xbsIndex_r4/Counter  cnt_type=Free Running  cnt_to=Inf  operation=Up  start_count=0  cnt_by_val=1  arith_type=Unsigned  n_bits=8  bin_pt=0  load_pin=off  rst=on  en=on  explicit_period=on  period=1  dbl_ovrd=off  use_behavioral_HDL=off  implementation=Fabric  block_type=counter
      settings: block_version=11.4
  sync_next_pps : Subsystem  Tag=xps:sw_reg  AncestorBlock=xps_library/software register  DataTypeOverride=Double  DataTypeOverrideAppliesTo=Fixed-point  MinMaxOverflowLogging=ForceOff  mask(swreg){mode=one value, io_dir=From Processor, io_delay=0, sample_period=1, names=reg, bitwidths=32, arith_types=0, bin_pts=[0], sim_port=on, show_format=off}
      mask prompts: io_dir "I/O direction"; io_delay "I/O delay"; sample_period "Sample period"; names "Name:"; bitwidths "Bitwidth:"; arith_types "Type (ufix=0, fix=1, bool=2):"; bin_pts "Binary pt:"; sim_port "Provide sim input/output?"; show_format "Print format string?"
      mask init:
      | swreg_init(gcb)
      settings: AttributesFormatString=1input
      mask TypeOptions mode: one value | fields of equal size | fields of arbitrary size
      mask Callback mode: swreg_cb(gcb);
      mask TypeOptions io_dir: To Processor | From Processor
      mask Callback io_dir:
      | mask_enables = get_param(gcb, 'MaskEnables');
      | mask_names = get_param(gcb, 'MaskNames');
      | if strcmp(get_param(gcb, 'io_dir'), 'To Processor'),
      |     mask_enables{ismember(mask_names, 'sample_period')} = 'off';
      | else
      |     mask_enables{ismember(mask_names, 'sample_period')} = 'on';
      | end
      | set_param(gcb, 'MaskEnables', mask_enables);
      mask Callback bitwidths:
      | swreg_maskcheck(gcb);
      | % blk = gcb;
      | % mode = get_param(blk, 'mode');
      | % current_widths = eval(get_param(blk, 'bitwidths'));
      | % if (strcmp(mode, 'one value') || strcmp(mode, 'fields of equal size')) && (length(current_widths) > 1),
      | %     error('Only one width may be specified for this mode.');
      | % elseif strcmp(mode, 'fields of arbitrary size')
      | %     current_names = textscan(strtrim(strrep(strrep(get_param(blk, 'names'), ']', ''), '[', '')), '%s');
      | %     current_names = current_names{1};
      | %     numios = length(current_names);
      | %     if length(current_widths) ~= numios,
      | %         error('%d field names specified, but %d widths?', numios, length(current_widths));
      | %     end
      | % end
      | % total_width = 0;
      | % for ctr = 1 : length(current_widths),
      | %     total_width = total_width + current_widths(ctr);
      | % end
      | % if total_width > 32,
      | %     error('Total width must be 32 or less, set to %d.', total_width);
      | % end
      mask Callback arith_types:
      | [numios, ~, ~, ~, current_types] = swreg_maskcheck(gcb);
      | % blk = gcb;
      | % mode = get_param(blk, 'mode');
      | % current_types = eval(get_param(blk, 'arith_types'));
      | % numios = length(current_types);
      | % if (strcmp(mode, 'one value') || strcmp(mode, 'fields of equal size')) && (length(current_types) > 1),
      | %     error('Only one type may be specified for this mode.');
      | % elseif strcmp(mode, 'fields of arbitrary size')
      | %     current_names = textscan(strtrim(strrep(strrep(get_param(blk, 'names'), ']', ''), '[', '')), '%s');
      | %     current_names = current_names{1};
      | %     numios = length(current_names);
      | %     if length(current_types) ~= numios,
      | %         error('%d field names specified, but %d types?', numios, length(current_types));
      | %     end
      | % end
      | problem = 0;
      | for ctr = 1 : numios,
      |     t = current_types(ctr);
      |     if (t < 0) || (t > 2),
      |         problem = t;
      |         ctr = numios + 1;
      |     end
      | end
      | if problem ~= 0,
      |     error('Type cannot be %i, must be 0, 1 or 2.', problem);
      | end
      mask Callback bin_pts:
      | swreg_maskcheck(gcb);
      | % blk = gcb;
      | % mode = get_param(blk, 'mode');
      | % current_bins = eval(get_param(blk, 'bin_pts'));
      | % if (strcmp(mode, 'one value') || strcmp(mode, 'fields of equal size')) && (length(current_bins) > 1),
      | %     error('Only one binary pt may be specified for this mode.');
      | % elseif strcmp(mode, 'fields of arbitrary size')
      | %     current_names = textscan(strtrim(strrep(strrep(get_param(blk, 'names'), ']', ''), '[', '')), '%s');
      | %     current_names = current_names{1};
      | %     numios = length(current_names);
      | %     if length(current_bins) ~= numios,
      | %         error('%d field names specified, but %d binary pts?', numios, length(current_bins));
      | %     end
      | % end
  sync_pulse_ : xbsIndex_r4/Gateway Out  inherit_from_input=off  hdl_port=on  timing_constraint=None  locs_specified=off  LOCs={}  UseAsDAC=off  DACChannel='1'  block_type=gatewayout
  tgbe0 : Subsystem  Tag=xps:tengbe_v2  AncestorBlock=xps_library/ten_Gbe_v2  mask(ten_GbE_v2){flavour=cx4, slot=1, port_r1=2, port_r2_cx4=0, port_r2_sfpp=0, rx_dist_ram=on, large_frames=off, show_param=on, pre_emph_r2=0.74, pre_emph=3, post_emph_r2=0.18, rxeqmix_r2=7, swing_r2=940, swing=800, fab_en=on, fab_mac=hex2dec('123456780000'), fab_ip=10*(2^24) + 0*(2^16) + 0*(2^8) + 2*(2^0), fab_udp=60001, fab_gate=1, cpu_rx_en=on, cpu_tx_en=on, ttl=hex2dec('FF'), promisc_mode=off, debug_ctr_width=16, txctr=on, txerrctr=off, txerrctr_len=4224, txofctr=on, txfullctr=off, txvldctr=on, txsnaplen=8192, rxctr=off, rxerrctr=off, rxerrctr_len=100, rxofctr=off, rxbadctr=off, rxvldctr=off, rxeofctr=off, rxsnaplen=0 - no snap}
      mask prompts: flavour "Mezzanine card flavour"; slot "Card slot"; port_r1 "Port"; port_r2_cx4 "Port"; port_r2_sfpp "Port"; rx_dist_ram "Shallow RX Fifo (Beware overruns!)"; large_frames "Enable Large TX Frames (8k+512)"; show_param "---------------------- Show Implementation Parameters -----------------------------------------------------------------------------------"; pre_emph_r2 "Pre-emphasis (dB)"; pre_emph "Pre-emphasis"; post_emph_r2 "Post-emphasis (dB)"; rxeqmix_r2 "Receive equalisation"; swing_r2 "Driver Swing Control (mVppd)"; swing "Differential swing"; fab_en "Enable fabric on startup"; fab_mac "Fabric MAC Address"; fab_ip "Fabric IP Address"; fab_udp "Fabric UDP Port"; fab_gate "Fabric Gateway"; cpu_rx_en "Enable CPU RX"; cpu_tx_en "Enable CPU TX"; promisc_mode "Promiscuous mode"; debug_ctr_width "Debug counter width"; txctr "TX - core_txctr"; txerrctr "TX packet length error - core_txerrctr"; txerrctr_len "-- expected TX packet length"; txofctr "TX overflow - core_txofctr"; txfullctr "TX full - core_txfullctr"; txvldctr "TX valid cycle - core_txvldctr"; txsnaplen "TX snapshot length"; rxctr "RX - core_rxctr"; rxerrctr "RX packet length error - core_rxerrctr"; rxerrctr_len "-- expected RX packet length"; rxofctr "RX overflow - core_rxofctr"; rxbadctr "RX bad - core_rxbadctr"; rxvldctr "RX valid cycle - core_rxvldctr"; rxeofctr "RX eof - core_rxeofctr"; rxsnaplen "RX snapshot length"
      mask help: This block sends and receives UDP frames (packets). It accepts a 64 bit wide data stream with user-determined frame breaks. The data stream is wrapped in a UDP frame for transmission. Incoming UDP packets are unwrapped and the data presented as a 64 bit wide stream.
      mask init:
      | temp = eval(get_param(gcb, 'debug_ctr_width'));
      | if temp <= 0,
      |     error('Debug counters cannot be ltoet zero.');
      | end
      | tengbe_v2_mask(gcb)
      mask TypeOptions flavour: sfp+ | cx4
      mask Callback flavour: tengbe_v2_callback
      mask TypeOptions slot: 0 | 1
      mask TypeOptions port_r1: 0 | 1 | 2 | 3
      mask TypeOptions port_r2_cx4: 0 | 1 | 2
      mask TypeOptions port_r2_sfpp: 0 | 1 | 2 | 3
      mask Callback show_param: tengbe_v2_callback
      mask TypeOptions pre_emph_r2: 0.15 | 0.3 | 0.45 | 0.61 | 0.74 | 0.91 | 1.07 | 1.25 | 1.36 | 1.55 | 1.74 | 1.94 | 2.11 | 2.32 | 2.54 | 2.77
      mask TypeOptions pre_emph: 0 | 1 | 2 | 3
      mask TypeOptions post_emph_r2: 0.18 | 0.19 | 0.2 | 0.39 | 0.63 | 0.82 | 1.07 | 1.32 | 1.6 | 1.65 | 1.94 | 2.21 | 2.52 | 2.76 | 3.08 | 3.41 | 3.77 | 3.97 | 4.36 | 4.73 | 5.16 | 5.47 | 5.93 | 6.38 | 6.89
      mask TypeOptions rxeqmix_r2: 0 | 1 | 2 | 3 | 4 | 5 | 6 | 7
      mask TypeOptions swing_r2: 110 | 210 | 310 | 400 | 480 | 570 | 660 | 740 | 810 | 880 | 940 | 990 | 1040 | 1080 | 1110 | 1130
      mask TypeOptions swing: 400 | 500 | 600 | 700 | 800
      mask Callback txerrctr:
      | blk = gcb;
      | mask_visibilities = get_param(blk, 'MaskVisibilities');
      | mask_names = get_param(blk, 'MaskNames');
      | if strcmp(get_param(blk, 'txerrctr'), 'on')
      |     mask_visibilities{ismember(mask_names, 'txerrctr_len')} = 'on';
      | else
      |     mask_visibilities{ismember(mask_names, 'txerrctr_len')} = 'off';
      | end
      | set_param(blk, 'MaskVisibilities', mask_visibilities);
      mask TypeOptions txsnaplen: 0 - no snap | 256 | 512 | 1024 | 2048 | 4096 | 8192 | 16384
      mask Callback rxerrctr:
      | blk = gcb;
      | mask_visibilities = get_param(blk, 'MaskVisibilities');
      | mask_names = get_param(blk, 'MaskNames');
      | if strcmp(get_param(blk, 'rxerrctr'), 'on')
      |     mask_visibilities{ismember(mask_names, 'rxerrctr_len')} = 'on';
      | else
      |     mask_visibilities{ismember(mask_names, 'rxerrctr_len')} = 'off';
      | end
      | set_param(blk, 'MaskVisibilities', mask_visibilities);
      mask TypeOptions rxsnaplen: 0 - no snap | 256 | 512 | 1024 | 2048 | 4096 | 8192 | 16384
  tgbe0_debug_reset : Subsystem  Tag=xps:sw_reg  AncestorBlock=xps_library/software register  mask(swreg){mode=one value, io_dir=From Processor, io_delay=0, sample_period=1, names=reg, bitwidths=32, arith_types=0, bin_pts=0, sim_port=on, show_format=off}
      mask prompts: io_dir "I/O direction"; io_delay "I/O delay"; sample_period "Sample period"; names "Name:"; bitwidths "Bitwidth:"; arith_types "Type (ufix=0, fix=1, bool=2):"; bin_pts "Binary pt:"; sim_port "Provide sim input/output?"; show_format "Print format string?"
      mask init:
      | swreg_init(gcb)
      settings: AttributesFormatString=1input
      mask TypeOptions mode: one value | fields of equal size | fields of arbitrary size
      mask Callback mode: swreg_cb(gcb);
      mask TypeOptions io_dir: To Processor | From Processor
      mask Callback io_dir:
      | mask_enables = get_param(gcb, 'MaskEnables');
      | mask_names = get_param(gcb, 'MaskNames');
      | if strcmp(get_param(gcb, 'io_dir'), 'To Processor'),
      |     mask_enables{ismember(mask_names, 'sample_period')} = 'off';
      | else
      |     mask_enables{ismember(mask_names, 'sample_period')} = 'on';
      | end
      | set_param(gcb, 'MaskEnables', mask_enables);
      mask Callback bitwidths: swreg_maskcheck(gcb);
      mask Callback arith_types: [numios, ~, ~, ~, current_types] = swreg_maskcheck(gcb);
      mask Callback bin_pts: swreg_maskcheck(gcb);
  tgbe0_dest_ip : Subsystem  Tag=xps:sw_reg  AncestorBlock=xps_library/software register  mask(swreg){mode=one value, io_dir=From Processor, io_delay=0, sample_period=1, names=reg, bitwidths=32, arith_types=0, bin_pts=0, sim_port=on, show_format=off}
      mask prompts: io_dir "I/O direction"; io_delay "I/O delay"; sample_period "Sample period"; names "Name:"; bitwidths "Bitwidth:"; arith_types "Type (ufix=0, fix=1, bool=2):"; bin_pts "Binary pt:"; sim_port "Provide sim input/output?"; show_format "Print format string?"
      mask init:
      | swreg_init(gcb)
      settings: AttributesFormatString=1input
      mask TypeOptions mode: one value | fields of equal size | fields of arbitrary size
      mask Callback mode: swreg_cb(gcb);
      mask TypeOptions io_dir: To Processor | From Processor
      mask Callback io_dir:
      | mask_enables = get_param(gcb, 'MaskEnables');
      | mask_names = get_param(gcb, 'MaskNames');
      | if strcmp(get_param(gcb, 'io_dir'), 'To Processor'),
      |     mask_enables{ismember(mask_names, 'sample_period')} = 'off';
      | else
      |     mask_enables{ismember(mask_names, 'sample_period')} = 'on';
      | end
      | set_param(gcb, 'MaskEnables', mask_enables);
      mask Callback bitwidths: swreg_maskcheck(gcb);
      mask Callback arith_types: [numios, ~, ~, ~, current_types] = swreg_maskcheck(gcb);
      mask Callback bin_pts: swreg_maskcheck(gcb);
  tgbe0_dest_port : Subsystem  Tag=xps:sw_reg  AncestorBlock=xps_library/software register  mask(swreg){mode=one value, io_dir=From Processor, io_delay=0, sample_period=1, names=reg, bitwidths=16, arith_types=0, bin_pts=0, sim_port=on, show_format=off}
      mask prompts: io_dir "I/O direction"; io_delay "I/O delay"; sample_period "Sample period"; names "Name:"; bitwidths "Bitwidth:"; arith_types "Type (ufix=0, fix=1, bool=2):"; bin_pts "Binary pt:"; sim_port "Provide sim input/output?"; show_format "Print format string?"
      mask init:
      | swreg_init(gcb)
      settings: AttributesFormatString=1input
      mask TypeOptions mode: one value | fields of equal size | fields of arbitrary size
      mask Callback mode: swreg_cb(gcb);
      mask TypeOptions io_dir: To Processor | From Processor
      mask Callback io_dir:
      | mask_enables = get_param(gcb, 'MaskEnables');
      | mask_names = get_param(gcb, 'MaskNames');
      | if strcmp(get_param(gcb, 'io_dir'), 'To Processor'),
      |     mask_enables{ismember(mask_names, 'sample_period')} = 'off';
      | else
      |     mask_enables{ismember(mask_names, 'sample_period')} = 'on';
      | end
      | set_param(gcb, 'MaskEnables', mask_enables);
      mask Callback bitwidths: swreg_maskcheck(gcb);
      mask Callback arith_types: [numios, ~, ~, ~, current_types] = swreg_maskcheck(gcb);
      mask Callback bin_pts: swreg_maskcheck(gcb);
  tgbe0_linkup : Subsystem  Tag=xps:sw_reg  AncestorBlock=xps_library/software register  mask(swreg){mode=one value, io_dir=To Processor, io_delay=0, sample_period=1, names=reg, bitwidths=1, arith_types=2, bin_pts=0, sim_port=on, show_format=off}
      mask prompts: io_dir "I/O direction"; io_delay "I/O delay"; sample_period "Sample period"; names "Name:"; bitwidths "Bitwidth:"; arith_types "Type (ufix=0, fix=1, bool=2):"; bin_pts "Binary pt:"; sim_port "Provide sim input/output?"; show_format "Print format string?"
      mask init:
      | swreg_init(gcb)
      settings: AttributesFormatString=1output
      mask TypeOptions mode: one value | fields of equal size | fields of arbitrary size
      mask Callback mode: swreg_cb(gcb);
      mask TypeOptions io_dir: To Processor | From Processor
      mask Callback io_dir:
      | mask_enables = get_param(gcb, 'MaskEnables');
      | mask_names = get_param(gcb, 'MaskNames');
      | if strcmp(get_param(gcb, 'io_dir'), 'To Processor'),
      |     mask_enables{ismember(mask_names, 'sample_period')} = 'off';
      | else
      |     mask_enables{ismember(mask_names, 'sample_period')} = 'on';
      | end
      | set_param(gcb, 'MaskEnables', mask_enables);
      mask Callback bitwidths:
      | swreg_maskcheck(gcb);
      | % blk = gcb;
      | % mode = get_param(blk, 'mode');
      | % current_widths = eval(get_param(blk, 'bitwidths'));
      | % if (strcmp(mode, 'one value') || strcmp(mode, 'fields of equal size')) && (length(current_widths) > 1),
      | %     error('Only one width may be specified for this mode.');
      | % elseif strcmp(mode, 'fields of arbitrary size')
      | %     current_names = textscan(strtrim(strrep(strrep(get_param(blk, 'names'), ']', ''), '[', '')), '%s');
      | %     current_names = current_names{1};
      | %     numios = length(current_names);
      | %     if length(current_widths) ~= numios,
      | %         error('%d field names specified, but %d widths?', numios, length(current_widths));
      | %     end
      | % end
      | % total_width = 0;
      | % for ctr = 1 : length(current_widths),
      | %     total_width = total_width + current_widths(ctr);
      | % end
      | % if total_width > 32,
      | %     error('Total width must be 32 or less, set to %d.', total_width);
      | % end
      mask Callback arith_types:
      | [numios, ~, ~, ~, current_types] = swreg_maskcheck(gcb);
      | % blk = gcb;
      | % mode = get_param(blk, 'mode');
      | % current_types = eval(get_param(blk, 'arith_types'));
      | % numios = length(current_types);
      | % if (strcmp(mode, 'one value') || strcmp(mode, 'fields of equal size')) && (length(current_types) > 1),
      | %     error('Only one type may be specified for this mode.');
      | % elseif strcmp(mode, 'fields of arbitrary size')
      | %     current_names = textscan(strtrim(strrep(strrep(get_param(blk, 'names'), ']', ''), '[', '')), '%s');
      | %     current_names = current_names{1};
      | %     numios = length(current_names);
      | %     if length(current_types) ~= numios,
      | %         error('%d field names specified, but %d types?', numios, length(current_types));
      | %     end
      | % end
      | problem = 0;
      | for ctr = 1 : numios,
      |     t = current_types(ctr);
      |     if (t < 0) || (t > 2),
      |         problem = t;
      |         ctr = numios + 1;
      |     end
      | end
      | if problem ~= 0,
      |     error('Type cannot be %i, must be 0, 1 or 2.', problem);
      | end
      mask Callback bin_pts:
      | swreg_maskcheck(gcb);
      | % blk = gcb;
      | % mode = get_param(blk, 'mode');
      | % current_bins = eval(get_param(blk, 'bin_pts'));
      | % if (strcmp(mode, 'one value') || strcmp(mode, 'fields of equal size')) && (length(current_bins) > 1),
      | %     error('Only one binary pt may be specified for this mode.');
      | % elseif strcmp(mode, 'fields of arbitrary size')
      | %     current_names = textscan(strtrim(strrep(strrep(get_param(blk, 'names'), ']', ''), '[', '')), '%s');
      | %     current_names = current_names{1};
      | %     numios = length(current_names);
      | %     if length(current_bins) ~= numios,
      | %         error('%d field names specified, but %d binary pts?', numios, length(current_bins));
      | %     end
      | % end
  tgbe0_tx : Subsystem  Tag=xps:sw_reg  AncestorBlock=xps_library/software register  mask(swreg){mode=one value, io_dir=To Processor, io_delay=0, sample_period=1, names=reg, bitwidths=1, arith_types=2, bin_pts=0, sim_port=on, show_format=off}
      mask prompts: io_dir "I/O direction"; io_delay "I/O delay"; sample_period "Sample period"; names "Name:"; bitwidths "Bitwidth:"; arith_types "Type (ufix=0, fix=1, bool=2):"; bin_pts "Binary pt:"; sim_port "Provide sim input/output?"; show_format "Print format string?"
      mask init:
      | swreg_init(gcb)
      settings: AttributesFormatString=1output
      mask TypeOptions mode: one value | fields of equal size | fields of arbitrary size
      mask Callback mode: swreg_cb(gcb);
      mask TypeOptions io_dir: To Processor | From Processor
      mask Callback io_dir:
      | mask_enables = get_param(gcb, 'MaskEnables');
      | mask_names = get_param(gcb, 'MaskNames');
      | if strcmp(get_param(gcb, 'io_dir'), 'To Processor'),
      |     mask_enables{ismember(mask_names, 'sample_period')} = 'off';
      | else
      |     mask_enables{ismember(mask_names, 'sample_period')} = 'on';
      | end
      | set_param(gcb, 'MaskEnables', mask_enables);
      mask Callback bitwidths:
      | swreg_maskcheck(gcb);
      | % blk = gcb;
      | % mode = get_param(blk, 'mode');
      | % current_widths = eval(get_param(blk, 'bitwidths'));
      | % if (strcmp(mode, 'one value') || strcmp(mode, 'fields of equal size')) && (length(current_widths) > 1),
      | %     error('Only one width may be specified for this mode.');
      | % elseif strcmp(mode, 'fields of arbitrary size')
      | %     current_names = textscan(strtrim(strrep(strrep(get_param(blk, 'names'), ']', ''), '[', '')), '%s');
      | %     current_names = current_names{1};
      | %     numios = length(current_names);
      | %     if length(current_widths) ~= numios,
      | %         error('%d field names specified, but %d widths?', numios, length(current_widths));
      | %     end
      | % end
      | % total_width = 0;
      | % for ctr = 1 : length(current_widths),
      | %     total_width = total_width + current_widths(ctr);
      | % end
      | % if total_width > 32,
      | %     error('Total width must be 32 or less, set to %d.', total_width);
      | % end
      mask Callback arith_types:
      | [numios, ~, ~, ~, current_types] = swreg_maskcheck(gcb);
      | % blk = gcb;
      | % mode = get_param(blk, 'mode');
      | % current_types = eval(get_param(blk, 'arith_types'));
      | % numios = length(current_types);
      | % if (strcmp(mode, 'one value') || strcmp(mode, 'fields of equal size')) && (length(current_types) > 1),
      | %     error('Only one type may be specified for this mode.');
      | % elseif strcmp(mode, 'fields of arbitrary size')
      | %     current_names = textscan(strtrim(strrep(strrep(get_param(blk, 'names'), ']', ''), '[', '')), '%s');
      | %     current_names = current_names{1};
      | %     numios = length(current_names);
      | %     if length(current_types) ~= numios,
      | %         error('%d field names specified, but %d types?', numios, length(current_types));
      | %     end
      | % end
      | problem = 0;
      | for ctr = 1 : numios,
      |     t = current_types(ctr);
      |     if (t < 0) || (t > 2),
      |         problem = t;
      |         ctr = numios + 1;
      |     end
      | end
      | if problem ~= 0,
      |     error('Type cannot be %i, must be 0, 1 or 2.', problem);
      | end
      mask Callback bin_pts:
      | swreg_maskcheck(gcb);
      | % blk = gcb;
      | % mode = get_param(blk, 'mode');
      | % current_bins = eval(get_param(blk, 'bin_pts'));
      | % if (strcmp(mode, 'one value') || strcmp(mode, 'fields of equal size')) && (length(current_bins) > 1),
      | %     error('Only one binary pt may be specified for this mode.');
      | % elseif strcmp(mode, 'fields of arbitrary size')
      | %     current_names = textscan(strtrim(strrep(strrep(get_param(blk, 'names'), ']', ''), '[', '')), '%s');
      | %     current_names = current_names{1};
      | %     numios = length(current_names);
      | %     if length(current_bins) ~= numios,
      | %         error('%d field names specified, but %d binary pts?', numios, length(current_bins));
      | %     end
      | % end
  tgbe0_tx_full : Subsystem  Tag=xps:sw_reg  AncestorBlock=xps_library/software register  mask(swreg){mode=one value, io_dir=To Processor, io_delay=0, sample_period=1, names=reg, bitwidths=1, arith_types=2, bin_pts=0, sim_port=on, show_format=off}
      mask prompts: io_dir "I/O direction"; io_delay "I/O delay"; sample_period "Sample period"; names "Name:"; bitwidths "Bitwidth:"; arith_types "Type (ufix=0, fix=1, bool=2):"; bin_pts "Binary pt:"; sim_port "Provide sim input/output?"; show_format "Print format string?"
      mask init:
      | swreg_init(gcb)
      settings: AttributesFormatString=1output
      mask TypeOptions mode: one value | fields of equal size | fields of arbitrary size
      mask Callback mode: swreg_cb(gcb);
      mask TypeOptions io_dir: To Processor | From Processor
      mask Callback io_dir:
      | mask_enables = get_param(gcb, 'MaskEnables');
      | mask_names = get_param(gcb, 'MaskNames');
      | if strcmp(get_param(gcb, 'io_dir'), 'To Processor'),
      |     mask_enables{ismember(mask_names, 'sample_period')} = 'off';
      | else
      |     mask_enables{ismember(mask_names, 'sample_period')} = 'on';
      | end
      | set_param(gcb, 'MaskEnables', mask_enables);
      mask Callback bitwidths:
      | swreg_maskcheck(gcb);
      | % blk = gcb;
      | % mode = get_param(blk, 'mode');
      | % current_widths = eval(get_param(blk, 'bitwidths'));
      | % if (strcmp(mode, 'one value') || strcmp(mode, 'fields of equal size')) && (length(current_widths) > 1),
      | %     error('Only one width may be specified for this mode.');
      | % elseif strcmp(mode, 'fields of arbitrary size')
      | %     current_names = textscan(strtrim(strrep(strrep(get_param(blk, 'names'), ']', ''), '[', '')), '%s');
      | %     current_names = current_names{1};
      | %     numios = length(current_names);
      | %     if length(current_widths) ~= numios,
      | %         error('%d field names specified, but %d widths?', numios, length(current_widths));
      | %     end
      | % end
      | % total_width = 0;
      | % for ctr = 1 : length(current_widths),
      | %     total_width = total_width + current_widths(ctr);
      | % end
      | % if total_width > 32,
      | %     error('Total width must be 32 or less, set to %d.', total_width);
      | % end
      mask Callback arith_types:
      | [numios, ~, ~, ~, current_types] = swreg_maskcheck(gcb);
      | % blk = gcb;
      | % mode = get_param(blk, 'mode');
      | % current_types = eval(get_param(blk, 'arith_types'));
      | % numios = length(current_types);
      | % if (strcmp(mode, 'one value') || strcmp(mode, 'fields of equal size')) && (length(current_types) > 1),
      | %     error('Only one type may be specified for this mode.');
      | % elseif strcmp(mode, 'fields of arbitrary size')
      | %     current_names = textscan(strtrim(strrep(strrep(get_param(blk, 'names'), ']', ''), '[', '')), '%s');
      | %     current_names = current_names{1};
      | %     numios = length(current_names);
      | %     if length(current_types) ~= numios,
      | %         error('%d field names specified, but %d types?', numios, length(current_types));
      | %     end
      | % end
      | problem = 0;
      | for ctr = 1 : numios,
      |     t = current_types(ctr);
      |     if (t < 0) || (t > 2),
      |         problem = t;
      |         ctr = numios + 1;
      |     end
      | end
      | if problem ~= 0,
      |     error('Type cannot be %i, must be 0, 1 or 2.', problem);
      | end
      mask Callback bin_pts:
      | swreg_maskcheck(gcb);
      | % blk = gcb;
      | % mode = get_param(blk, 'mode');
      | % current_bins = eval(get_param(blk, 'bin_pts'));
      | % if (strcmp(mode, 'one value') || strcmp(mode, 'fields of equal size')) && (length(current_bins) > 1),
      | %     error('Only one binary pt may be specified for this mode.');
      | % elseif strcmp(mode, 'fields of arbitrary size')
      | %     current_names = textscan(strtrim(strrep(strrep(get_param(blk, 'names'), ']', ''), '[', '')), '%s');
      | %     current_names = current_names{1};
      | %     numios = length(current_names);
      | %     if length(current_bins) ~= numios,
      | %         error('%d field names specified, but %d binary pts?', numios, length(current_bins));
      | %     end
      | % end
  tgbe0_tx_of : Subsystem  Tag=xps:sw_reg  AncestorBlock=xps_library/software register  mask(swreg){mode=one value, io_dir=To Processor, io_delay=0, sample_period=1, names=reg, bitwidths=1, arith_types=2, bin_pts=0, sim_port=on, show_format=off}
      mask prompts: io_dir "I/O direction"; io_delay "I/O delay"; sample_period "Sample period"; names "Name:"; bitwidths "Bitwidth:"; arith_types "Type (ufix=0, fix=1, bool=2):"; bin_pts "Binary pt:"; sim_port "Provide sim input/output?"; show_format "Print format string?"
      mask init:
      | swreg_init(gcb)
      settings: AttributesFormatString=1output
      mask TypeOptions mode: one value | fields of equal size | fields of arbitrary size
      mask Callback mode: swreg_cb(gcb);
      mask TypeOptions io_dir: To Processor | From Processor
      mask Callback io_dir:
      | mask_enables = get_param(gcb, 'MaskEnables');
      | mask_names = get_param(gcb, 'MaskNames');
      | if strcmp(get_param(gcb, 'io_dir'), 'To Processor'),
      |     mask_enables{ismember(mask_names, 'sample_period')} = 'off';
      | else
      |     mask_enables{ismember(mask_names, 'sample_period')} = 'on';
      | end
      | set_param(gcb, 'MaskEnables', mask_enables);
      mask Callback bitwidths:
      | swreg_maskcheck(gcb);
      | % blk = gcb;
      | % mode = get_param(blk, 'mode');
      | % current_widths = eval(get_param(blk, 'bitwidths'));
      | % if (strcmp(mode, 'one value') || strcmp(mode, 'fields of equal size')) && (length(current_widths) > 1),
      | %     error('Only one width may be specified for this mode.');
      | % elseif strcmp(mode, 'fields of arbitrary size')
      | %     current_names = textscan(strtrim(strrep(strrep(get_param(blk, 'names'), ']', ''), '[', '')), '%s');
      | %     current_names = current_names{1};
      | %     numios = length(current_names);
      | %     if length(current_widths) ~= numios,
      | %         error('%d field names specified, but %d widths?', numios, length(current_widths));
      | %     end
      | % end
      | % total_width = 0;
      | % for ctr = 1 : length(current_widths),
      | %     total_width = total_width + current_widths(ctr);
      | % end
      | % if total_width > 32,
      | %     error('Total width must be 32 or less, set to %d.', total_width);
      | % end
      mask Callback arith_types:
      | [numios, ~, ~, ~, current_types] = swreg_maskcheck(gcb);
      | % blk = gcb;
      | % mode = get_param(blk, 'mode');
      | % current_types = eval(get_param(blk, 'arith_types'));
      | % numios = length(current_types);
      | % if (strcmp(mode, 'one value') || strcmp(mode, 'fields of equal size')) && (length(current_types) > 1),
      | %     error('Only one type may be specified for this mode.');
      | % elseif strcmp(mode, 'fields of arbitrary size')
      | %     current_names = textscan(strtrim(strrep(strrep(get_param(blk, 'names'), ']', ''), '[', '')), '%s');
      | %     current_names = current_names{1};
      | %     numios = length(current_names);
      | %     if length(current_types) ~= numios,
      | %         error('%d field names specified, but %d types?', numios, length(current_types));
      | %     end
      | % end
      | problem = 0;
      | for ctr = 1 : numios,
      |     t = current_types(ctr);
      |     if (t < 0) || (t > 2),
      |         problem = t;
      |         ctr = numios + 1;
      |     end
      | end
      | if problem ~= 0,
      |     error('Type cannot be %i, must be 0, 1 or 2.', problem);
      | end
      mask Callback bin_pts:
      | swreg_maskcheck(gcb);
      | % blk = gcb;
      | % mode = get_param(blk, 'mode');
      | % current_bins = eval(get_param(blk, 'bin_pts'));
      | % if (strcmp(mode, 'one value') || strcmp(mode, 'fields of equal size')) && (length(current_bins) > 1),
      | %     error('Only one binary pt may be specified for this mode.');
      | % elseif strcmp(mode, 'fields of arbitrary size')
      | %     current_names = textscan(strtrim(strrep(strrep(get_param(blk, 'names'), ']', ''), '[', '')), '%s');
      | %     current_names = current_names{1};
      | %     numios = length(current_names);
      | %     if length(current_bins) ~= numios,
      | %         error('%d field names specified, but %d binary pts?', numios, length(current_bins));
      | %     end
      | % end
  time_lsb : Subsystem  Tag=xps:sw_reg  AncestorBlock=xps_library/software register  DataTypeOverride=Double  DataTypeOverrideAppliesTo=Fixed-point  MinMaxOverflowLogging=ForceOff  mask(swreg){mode=one value, io_dir=From Processor, io_delay=0, sample_period=1, names=reg, bitwidths=32, arith_types=0, bin_pts=[0], sim_port=on, show_format=off}
      mask prompts: io_dir "I/O direction"; io_delay "I/O delay"; sample_period "Sample period"; names "Name:"; bitwidths "Bitwidth:"; arith_types "Type (ufix=0, fix=1, bool=2):"; bin_pts "Binary pt:"; sim_port "Provide sim input/output?"; show_format "Print format string?"
      mask init:
      | swreg_init(gcb)
      settings: AttributesFormatString=1input
      mask TypeOptions mode: one value | fields of equal size | fields of arbitrary size
      mask Callback mode: swreg_cb(gcb);
      mask TypeOptions io_dir: To Processor | From Processor
      mask Callback io_dir:
      | mask_enables = get_param(gcb, 'MaskEnables');
      | mask_names = get_param(gcb, 'MaskNames');
      | if strcmp(get_param(gcb, 'io_dir'), 'To Processor'),
      |     mask_enables{ismember(mask_names, 'sample_period')} = 'off';
      | else
      |     mask_enables{ismember(mask_names, 'sample_period')} = 'on';
      | end
      | set_param(gcb, 'MaskEnables', mask_enables);
      mask Callback bitwidths:
      | swreg_maskcheck(gcb);
      | % blk = gcb;
      | % mode = get_param(blk, 'mode');
      | % current_widths = eval(get_param(blk, 'bitwidths'));
      | % if (strcmp(mode, 'one value') || strcmp(mode, 'fields of equal size')) && (length(current_widths) > 1),
      | %     error('Only one width may be specified for this mode.');
      | % elseif strcmp(mode, 'fields of arbitrary size')
      | %     current_names = textscan(strtrim(strrep(strrep(get_param(blk, 'names'), ']', ''), '[', '')), '%s');
      | %     current_names = current_names{1};
      | %     numios = length(current_names);
      | %     if length(current_widths) ~= numios,
      | %         error('%d field names specified, but %d widths?', numios, length(current_widths));
      | %     end
      | % end
      | % total_width = 0;
      | % for ctr = 1 : length(current_widths),
      | %     total_width = total_width + current_widths(ctr);
      | % end
      | % if total_width > 32,
      | %     error('Total width must be 32 or less, set to %d.', total_width);
      | % end
      mask Callback arith_types:
      | [numios, ~, ~, ~, current_types] = swreg_maskcheck(gcb);
      | % blk = gcb;
      | % mode = get_param(blk, 'mode');
      | % current_types = eval(get_param(blk, 'arith_types'));
      | % numios = length(current_types);
      | % if (strcmp(mode, 'one value') || strcmp(mode, 'fields of equal size')) && (length(current_types) > 1),
      | %     error('Only one type may be specified for this mode.');
      | % elseif strcmp(mode, 'fields of arbitrary size')
      | %     current_names = textscan(strtrim(strrep(strrep(get_param(blk, 'names'), ']', ''), '[', '')), '%s');
      | %     current_names = current_names{1};
      | %     numios = length(current_names);
      | %     if length(current_types) ~= numios,
      | %         error('%d field names specified, but %d types?', numios, length(current_types));
      | %     end
      | % end
      | problem = 0;
      | for ctr = 1 : numios,
      |     t = current_types(ctr);
      |     if (t < 0) || (t > 2),
      |         problem = t;
      |         ctr = numios + 1;
      |     end
      | end
      | if problem ~= 0,
      |     error('Type cannot be %i, must be 0, 1 or 2.', problem);
      | end
      mask Callback bin_pts:
      | swreg_maskcheck(gcb);
      | % blk = gcb;
      | % mode = get_param(blk, 'mode');
      | % current_bins = eval(get_param(blk, 'bin_pts'));
      | % if (strcmp(mode, 'one value') || strcmp(mode, 'fields of equal size')) && (length(current_bins) > 1),
      | %     error('Only one binary pt may be specified for this mode.');
      | % elseif strcmp(mode, 'fields of arbitrary size')
      | %     current_names = textscan(strtrim(strrep(strrep(get_param(blk, 'names'), ']', ''), '[', '')), '%s');
      | %     current_names = current_names{1};
      | %     numios = length(current_names);
      | %     if length(current_bins) ~= numios,
      | %         error('%d field names specified, but %d binary pts?', numios, length(current_bins));
      | %     end
      | % end
  time_msb : Subsystem  Tag=xps:sw_reg  AncestorBlock=xps_library/software register  DataTypeOverride=Double  DataTypeOverrideAppliesTo=Fixed-point  MinMaxOverflowLogging=ForceOff  mask(swreg){mode=one value, io_dir=From Processor, io_delay=0, sample_period=1, names=reg, bitwidths=32, arith_types=0, bin_pts=[0], sim_port=on, show_format=off}
      mask prompts: io_dir "I/O direction"; io_delay "I/O delay"; sample_period "Sample period"; names "Name:"; bitwidths "Bitwidth:"; arith_types "Type (ufix=0, fix=1, bool=2):"; bin_pts "Binary pt:"; sim_port "Provide sim input/output?"; show_format "Print format string?"
      mask init:
      | swreg_init(gcb)
      settings: AttributesFormatString=1input
      mask TypeOptions mode: one value | fields of equal size | fields of arbitrary size
      mask Callback mode: swreg_cb(gcb);
      mask TypeOptions io_dir: To Processor | From Processor
      mask Callback io_dir:
      | mask_enables = get_param(gcb, 'MaskEnables');
      | mask_names = get_param(gcb, 'MaskNames');
      | if strcmp(get_param(gcb, 'io_dir'), 'To Processor'),
      |     mask_enables{ismember(mask_names, 'sample_period')} = 'off';
      | else
      |     mask_enables{ismember(mask_names, 'sample_period')} = 'on';
      | end
      | set_param(gcb, 'MaskEnables', mask_enables);
      mask Callback bitwidths:
      | swreg_maskcheck(gcb);
      | % blk = gcb;
      | % mode = get_param(blk, 'mode');
      | % current_widths = eval(get_param(blk, 'bitwidths'));
      | % if (strcmp(mode, 'one value') || strcmp(mode, 'fields of equal size')) && (length(current_widths) > 1),
      | %     error('Only one width may be specified for this mode.');
      | % elseif strcmp(mode, 'fields of arbitrary size')
      | %     current_names = textscan(strtrim(strrep(strrep(get_param(blk, 'names'), ']', ''), '[', '')), '%s');
      | %     current_names = current_names{1};
      | %     numios = length(current_names);
      | %     if length(current_widths) ~= numios,
      | %         error('%d field names specified, but %d widths?', numios, length(current_widths));
      | %     end
      | % end
      | % total_width = 0;
      | % for ctr = 1 : length(current_widths),
      | %     total_width = total_width + current_widths(ctr);
      | % end
      | % if total_width > 32,
      | %     error('Total width must be 32 or less, set to %d.', total_width);
      | % end
      mask Callback arith_types:
      | [numios, ~, ~, ~, current_types] = swreg_maskcheck(gcb);
      | % blk = gcb;
      | % mode = get_param(blk, 'mode');
      | % current_types = eval(get_param(blk, 'arith_types'));
      | % numios = length(current_types);
      | % if (strcmp(mode, 'one value') || strcmp(mode, 'fields of equal size')) && (length(current_types) > 1),
      | %     error('Only one type may be specified for this mode.');
      | % elseif strcmp(mode, 'fields of arbitrary size')
      | %     current_names = textscan(strtrim(strrep(strrep(get_param(blk, 'names'), ']', ''), '[', '')), '%s');
      | %     current_names = current_names{1};
      | %     numios = length(current_names);
      | %     if length(current_types) ~= numios,
      | %         error('%d field names specified, but %d types?', numios, length(current_types));
      | %     end
      | % end
      | problem = 0;
      | for ctr = 1 : numios,
      |     t = current_types(ctr);
      |     if (t < 0) || (t > 2),
      |         problem = t;
      |         ctr = numios + 1;
      |     end
      | end
      | if problem ~= 0,
      |     error('Type cannot be %i, must be 0, 1 or 2.', problem);
      | end
      mask Callback bin_pts:
      | swreg_maskcheck(gcb);
      | % blk = gcb;
      | % mode = get_param(blk, 'mode');
      | % current_bins = eval(get_param(blk, 'bin_pts'));
      | % if (strcmp(mode, 'one value') || strcmp(mode, 'fields of equal size')) && (length(current_bins) > 1),
      | %     error('Only one binary pt may be specified for this mode.');
      | % elseif strcmp(mode, 'fields of arbitrary size')
      | %     current_names = textscan(strtrim(strrep(strrep(get_param(blk, 'names'), ']', ''), '[', '')), '%s');
      | %     current_names = current_names{1};
      | %     numios = length(current_names);
      | %     if length(current_bins) ~= numios,
      | %         error('%d field names specified, but %d binary pts?', numios, length(current_bins));
      | %     end
      | % end
  timestamp_ : xbsIndex_r4/Gateway Out  inherit_from_input=off  hdl_port=on  timing_constraint=None  locs_specified=off  LOCs={}  UseAsDAC=off  DACChannel='1'  block_type=gatewayout
  upper_adc_threshold : Subsystem  Tag=xps:sw_reg  AncestorBlock=xps_library/software register  DataTypeOverride=Double  DataTypeOverrideAppliesTo=Fixed-point  MinMaxOverflowLogging=ForceOff  mask(swreg){mode=one value, io_dir=From Processor, io_delay=0, sample_period=1, names=reg, bitwidths=32, arith_types=0, bin_pts=[0], sim_port=off, show_format=off}
      mask prompts: io_dir "I/O direction"; io_delay "I/O delay"; sample_period "Sample period"; names "Name:"; bitwidths "Bitwidth:"; arith_types "Type (ufix=0, fix=1, bool=2):"; bin_pts "Binary pt:"; sim_port "Provide sim input/output?"; show_format "Print format string?"
      mask init:
      | swreg_init(gcb)
      settings: AttributesFormatString=1input
      mask TypeOptions mode: one value | fields of equal size | fields of arbitrary size
      mask Callback mode: swreg_cb(gcb);
      mask TypeOptions io_dir: To Processor | From Processor
      mask Callback io_dir:
      | mask_enables = get_param(gcb, 'MaskEnables');
      | mask_names = get_param(gcb, 'MaskNames');
      | if strcmp(get_param(gcb, 'io_dir'), 'To Processor'),
      |     mask_enables{ismember(mask_names, 'sample_period')} = 'off';
      | else
      |     mask_enables{ismember(mask_names, 'sample_period')} = 'on';
      | end
      | set_param(gcb, 'MaskEnables', mask_enables);
      mask Callback bitwidths:
      | swreg_maskcheck(gcb);
      | % blk = gcb;
      | % mode = get_param(blk, 'mode');
      | % current_widths = eval(get_param(blk, 'bitwidths'));
      | % if (strcmp(mode, 'one value') || strcmp(mode, 'fields of equal size')) && (length(current_widths) > 1),
      | %     error('Only one width may be specified for this mode.');
      | % elseif strcmp(mode, 'fields of arbitrary size')
      | %     current_names = textscan(strtrim(strrep(strrep(get_param(blk, 'names'), ']', ''), '[', '')), '%s');
      | %     current_names = current_names{1};
      | %     numios = length(current_names);
      | %     if length(current_widths) ~= numios,
      | %         error('%d field names specified, but %d widths?', numios, length(current_widths));
      | %     end
      | % end
      | % total_width = 0;
      | % for ctr = 1 : length(current_widths),
      | %     total_width = total_width + current_widths(ctr);
      | % end
      | % if total_width > 32,
      | %     error('Total width must be 32 or less, set to %d.', total_width);
      | % end
      mask Callback arith_types:
      | [numios, ~, ~, ~, current_types] = swreg_maskcheck(gcb);
      | % blk = gcb;
      | % mode = get_param(blk, 'mode');
      | % current_types = eval(get_param(blk, 'arith_types'));
      | % numios = length(current_types);
      | % if (strcmp(mode, 'one value') || strcmp(mode, 'fields of equal size')) && (length(current_types) > 1),
      | %     error('Only one type may be specified for this mode.');
      | % elseif strcmp(mode, 'fields of arbitrary size')
      | %     current_names = textscan(strtrim(strrep(strrep(get_param(blk, 'names'), ']', ''), '[', '')), '%s');
      | %     current_names = current_names{1};
      | %     numios = length(current_names);
      | %     if length(current_types) ~= numios,
      | %         error('%d field names specified, but %d types?', numios, length(current_types));
      | %     end
      | % end
      | problem = 0;
      | for ctr = 1 : numios,
      |     t = current_types(ctr);
      |     if (t < 0) || (t > 2),
      |         problem = t;
      |         ctr = numios + 1;
      |     end
      | end
      | if problem ~= 0,
      |     error('Type cannot be %i, must be 0, 1 or 2.', problem);
      | end
      mask Callback bin_pts:
      | swreg_maskcheck(gcb);
      | % blk = gcb;
      | % mode = get_param(blk, 'mode');
      | % current_bins = eval(get_param(blk, 'bin_pts'));
      | % if (strcmp(mode, 'one value') || strcmp(mode, 'fields of equal size')) && (length(current_bins) > 1),
      | %     error('Only one binary pt may be specified for this mode.');
      | % elseif strcmp(mode, 'fields of arbitrary size')
      | %     current_names = textscan(strtrim(strrep(strrep(get_param(blk, 'names'), ']', ''), '[', '')), '%s');
      | %     current_names = current_names{1};
      | %     numios = length(current_names);
      | %     if length(current_bins) ~= numios,
      | %         error('%d field names specified, but %d binary pts?', numios, length(current_bins));
      | %     end
      | % end
  usec_tick_ : xbsIndex_r4/Gateway Out  inherit_from_input=off  hdl_port=on  timing_constraint=None  locs_specified=off  LOCs={}  UseAsDAC=off  DACChannel='1'  block_type=gatewayout
  wait_for_pps_ : xbsIndex_r4/Gateway Out  inherit_from_input=off  hdl_port=on  timing_constraint=None  locs_specified=off  LOCs={}  UseAsDAC=off  DACChannel='1'  block_type=gatewayout
  window_size : xbsIndex_r4/Constant  const=1024/2  gui_display_data_type=Fixed-point  arith_type=Signed (2's comp)  n_bits=16  bin_pt=0  preci_type=Single  exp_width=8  frac_width=24  explicit_period=off  period=1  equ=P=C  opselect=C  inp2=PCIN>>17  opr=+  inp1=P  carry=CIN  dbl_ovrd=off  block_type=constant
  window_size1 : xbsIndex_r4/Constant  const=200  gui_display_data_type=Fixed-point  arith_type=Unsigned  n_bits=32  bin_pt=0  preci_type=Single  exp_width=8  frac_width=24  explicit_period=off  period=1  equ=P=C  opselect=C  inp2=PCIN>>17  opr=+  inp1=P  carry=CIN  dbl_ovrd=off  block_type=constant
  xsg_core_config : xps_library/XSG core config  Tag=xps:xsg  hw_sys=ROACH:sx95t  clk_src=adc0_clk  ROACH_clk_src=adc0_clk  ROACH2_clk_src=sys_clk  MKDIG_clk_src=sys_clk  clk_rate=200  sample_period=1  synthesis_tool=XST
  wires:
  Band-Limited White Noise/1 -> Sum/2
  Sine Wave/1 -> Sum/1
  Pulse Generator/1 -> katadc/3(sim_sync)
  Constant5/1 -> katadc/4(sim_data_valid)
  Sum/1 -> katadc/2(sim_data1), katadc/1(sim_data0)
  katadc/1(data0_0) -> Delay179/1
  katadc/2(data0_1) -> Delay180/1
  katadc/3(data0_2) -> Delay181/1
  katadc/4(data0_3) -> Delay182/1
  katadc/6(data1_0) -> Delay184/1
  katadc/7(data1_1) -> Delay185/1
  katadc/8(data1_2) -> Delay186/1
  katadc/9(data1_3) -> Delay187/1
  Delay54/1 -> pfb_fir_real/2(pol1_in1)
  Delay55/1 -> pfb_fir_real/3(pol1_in2)
  Delay198/1 -> pfb_fir_real/4(pol1_in3)
  Delay249/1 -> pfb_fir_real/5(pol1_in4)
  Delay253/1 -> pfb_fir_real/9(pol2_in4)
  Delay252/1 -> pfb_fir_real/8(pol2_in3)
  Delay251/1 -> pfb_fir_real/7(pol2_in2)
  Delay250/1 -> pfb_fir_real/6(pol2_in1)
  katadc/11(sync0) -> Delay189/1
  katadc/12(sync1) -> Delay190/1
  katadc/13(sync2) -> Delay191/1
  katadc/14(sync3) -> Delay192/1
  pfb_fir_real/1(sync_out) -> Delay90/1
  coarse_fft_shift_mask/1(in_reg) -> Delay35/1
  Constant6/1 -> coarse_fft_shift_mask/1(sim_1)
  err_clear_sim4/1 -> tgbe0_dest_port/1(sim_1)
  tgbe0_dest_port/1(in_reg) -> Delay38/1
  err_clear_sim3/1 -> tgbe0_dest_ip/1(sim_1)
  tgbe0_dest_ip/1(in_reg) -> Delay37/1
  packetizer/3(data_valid) -> [packetiser_dout_v]
  Constant9/1 -> tgbe0/7(rx_ack), tgbe0/8(rx_overrun_ack)
  tgbe0/6(rx_data) -> Terminator5/1
  tgbe0/7(rx_valid) -> Terminator6/1
  tgbe0/8(rx_source_ip) -> Terminator7/1
  tgbe0/9(rx_source_port) -> Terminator8/1
  tgbe0/10(rx_end_of_frame) -> Terminator9/1
  tgbe0/11(rx_bad_frame) -> Terminator10/1
  posedge1/1(out) -> Logical8/1, [eth_eof]
  accumulation_length/1(in_reg) -> Delay36/1
  accumlation_count/1 -> accumulation_length/1(sim_1)
  Relational1/1 -> Logical6/2, Logical3/1
  Concat2/1 -> Concat3/1
  simple_bram_vacc_i_even/2(valid) -> Delay83/1
  simple_bram_vacc_q_even/2(valid) -> Delay106/1
  simple_bram_vacc_u_even/2(valid) -> Delay129/1
  simple_bram_vacc_v_even/2(valid) -> Delay131/1
  Logical2/1 -> Logical5/1
  katadc/10(or1) -> Delay188/1
  katadc/5(or0) -> Delay183/1
  simple_bram_vacc_i_even/1(dout) -> Delay59/1
  simple_bram_vacc_q_even/1(dout) -> Delay105/1
  simple_bram_vacc_u_even/1(dout) -> Delay128/1
  simple_bram_vacc_v_even/1(dout) -> Delay130/1
  Counter1/1 -> [clk_cnt], Relational3/1
  window_size/1 -> Relational3/2
  Relational3/1 -> posedge2/1(in), Logical1/1
  posedge2/1(out) -> Delay147/1
  [stokes_sync_out] -> Delay10/1, Logical3/2, Logical1/2
  Logical1/1 -> Counter1/1
  Logical3/1 -> Counter2/1
  Concat1/1 -> Concat3/2
  simple_bram_vacc_i_odd/2(valid) -> Delay133/1
  simple_bram_vacc_q_odd/2(valid) -> Delay135/1
  simple_bram_vacc_u_odd/2(valid) -> Delay137/1
  simple_bram_vacc_v_odd/2(valid) -> Delay139/1
  Logical4/1 -> Logical5/2
  simple_bram_vacc_i_odd/1(dout) -> Delay132/1
  simple_bram_vacc_q_odd/1(dout) -> Delay134/1
  simple_bram_vacc_u_odd/1(dout) -> Delay136/1
  simple_bram_vacc_v_odd/1(dout) -> Delay138/1
  Concat3/1 -> Delay28/1
  Logical6/1 -> posedge/1(in)
  Delay10/1 -> Logical6/1
  tgbe0/1(led_up) -> [eth_up], Delay32/1
  tgbe0/2(led_rx) -> Terminator20/1
  tgbe0/3(led_tx) -> Delay31/1
  Delay13/1 -> simple_bram_vacc_q_even/1(new_acc)
  Delay14/1 -> simple_bram_vacc_u_even/1(new_acc)
  Delay15/1 -> simple_bram_vacc_v_even/1(new_acc)
  Delay16/1 -> simple_bram_vacc_i_odd/1(new_acc)
  Delay17/1 -> simple_bram_vacc_q_odd/1(new_acc)
  Delay18/1 -> simple_bram_vacc_u_odd/1(new_acc)
  Delay19/1 -> simple_bram_vacc_v_odd/1(new_acc)
  Delay20/1 -> simple_bram_vacc_v_odd/2(din)
  Delay21/1 -> simple_bram_vacc_u_odd/2(din)
  Delay22/1 -> simple_bram_vacc_q_odd/2(din)
  Delay23/1 -> simple_bram_vacc_i_odd/2(din)
  Delay24/1 -> simple_bram_vacc_v_even/2(din)
  Delay25/1 -> simple_bram_vacc_u_even/2(din)
  Delay26/1 -> simple_bram_vacc_q_even/2(din)
  Delay11/1 -> tgbe0_tx_of/1(out_reg)
  Delay30/1 -> tgbe0_tx_full/1(out_reg)
  Delay31/1 -> tgbe0_tx/1(out_reg)
  Delay32/1 -> tgbe0_linkup/1(out_reg)
  Delay33/1 -> tgbe0/1(rst)
  Delay12/1 -> simple_bram_vacc_i_even/1(new_acc)
  accumulation_cnt/1(sim_out) -> Terminator1/1
  Delay34/1 -> Slice1/1, accumulation_cnt/1(out_reg)
  Delay35/1 -> fft_wideband_real/2(shift)
  Delay36/1 -> Relational1/2
  Delay37/1 -> tgbe0/4(tx_dest_ip)
  Delay38/1 -> tgbe0/5(tx_dest_port)
  Counter3/1 -> Delay8/1, Delay40/1
  eth_eof_cnt/1(sim_out) -> Terminator3/1
  Delay40/1 -> eth_eof_cnt/1(out_reg)
  Delay41/1 -> Counter3/2
  Counter2/1 -> Relational1/1, Delay34/1
  Signal Builder/1(Signal 1) -> eth_reset/1(sim_1)
  eth_reset/1(in_reg) -> Slice/1
  [eth_reset] -> Delay53/1
  Delay53/1 -> Counter3/1
  Delay56/1 -> pfb_fir_real/1(sync)
  Delay28/1 -> packetizer/2(din)
  manual_sync/1(in_reg) -> Slice2/1
  Constant8/1 -> manual_sync/1(sim_1)
  Slice2/1 -> posedge5/1(in)
  packetiser_din_v_cnt/1(sim_out) -> Terminator28/1
  Counter8/1 -> [packetiser_dint_v_cnt], Delay72/1
  Logical5/1 -> Delay29/1, Delay69/1, [packetiser_din_v]
  Delay69/1 -> Counter8/2
  packetiser_dout_v_cnt/1(sim_out) -> Terminator29/1
  Counter9/1 -> [packetiser_dout_v_cnt], Delay71/1
  [packetiser_dout_v] -> Delay70/1
  Delay70/1 -> Counter9/2
  acc_trig_cnt/1(sim_out) -> Terminator30/1
  Counter10/1 -> acc_trig_cnt/1(out_reg)
  posedge10/1(out) -> Counter10/1
  [acc_trig] -> posedge10/1(in)
  Counter11/1 -> [packet_length_cnt], Relational2/1
  Logical8/1 -> Counter11/1
  [queue_empty] -> Inverter2/1
  Mux/1 -> [eth_tx_data], tgbe0/2(tx_data)
  Logical20/1 -> Delay49/1
  packetizer/4(buffer_overflow) -> [packetiser_of]
  [packetiser_din_v] -> posedge11/1(in)
  [eth_reset] -> posedge13/1(in)
  Logical9/1 -> Counter12/1
  posedge12/1(out) -> Counter12/2
  Delay29/1 -> packetizer/1(din_valid)
  Counter12/1 -> Slice6/1
  Slice6/1 -> Logical10/1
  Logical10/1 -> Delay177/1
  Inverter/1 -> Logical9/2
  tgbe0_linkup/1(sim_out) -> Terminator2/1
  tgbe0_tx/1(sim_out) -> Terminator4/1
  tgbe0_tx_full/1(sim_out) -> Terminator11/1
  tgbe0_tx_of/1(sim_out) -> Terminator17/1
  Delay68/1 -> Inverter/1, Logical10/2, posedge12/1(in)
  Delay71/1 -> packetiser_dout_v_cnt/1(out_reg)
  Delay72/1 -> packetiser_din_v_cnt/1(out_reg)
  packetiser_of_cnt/1(sim_out) -> Terminator18/1
  Delay74/1 -> packetiser_of_cnt/1(out_reg)
  posedge13/1(out) -> Delay33/1
  [eth_reset] -> Delay73/1
  Delay73/1 -> Counter8/1
  [eth_reset] -> Delay75/1
  Delay75/1 -> Counter9/1
  err_clear_sim1/1 -> tgbe0_debug_reset/1(sim_1)
  tgbe0_debug_reset/1(in_reg) -> Delay78/1
  Delay78/1 -> Slice7/1
  Slice7/1 -> tgbe0/9(debug_rst)
  tgbe0/12(rx_overrun) -> Terminator19/1
  Delay84/1 -> [pfb_sync_out], fft_wideband_real/1(sync)
  packetiser_perc_full/1(sim_out) -> Terminator12/1
  [packetiser_perc_full] -> Delay104/1
  Delay104/1 -> packetiser_perc_full/1(out_reg)
  packetizer/2(data_sout) -> [packetiser_dout]
  packetizer/1(data_addr) -> [packetiser_addr]
  [acc_trig] -> Delay12/1
  [acc_trig] -> Delay13/1
  [acc_trig] -> Delay14/1
  [acc_trig] -> Delay15/1
  [acc_trig] -> Delay16/1
  [acc_trig] -> Delay17/1
  [acc_trig] -> Delay18/1
  [acc_trig] -> Delay19/1
  [packetiser_dout_v] -> Delay113/1
  [packetiser_dout] -> Delay112/1
  Delay112/1 -> FIFO/1
  Delay113/1 -> FIFO/2
  Delay114/1 -> FIFO/4
  [eth_reset] -> Delay114/1
  [eth_eof] -> Delay94/1
  [eth_eof] -> Delay41/1
  [eth_data_tx_valid] -> FIFO/3
  FIFO/2 -> [queue_empty]
  [eth_reset] -> Logical8/2
  FIFO/4 -> [queue_full]
  FIFO/1 -> [queue_dout]
  Counter13/1 -> [interpacket_length_cnt], Relational4/1
  Logical11/1 -> Counter13/1
  Delay116/1 -> Slice16/1
  Relational4/1 -> posedge14/1(in)
  [eth_reset] -> Logical11/2
  eth_interframe_length_/1 -> eth_interpacket_length/1(sim_1)
  eth_interpacket_length/1(in_reg) -> Delay116/1
  Logical12/1 -> Counter11/2, [eth_data_tx_valid]
  Counter14/1 -> Slice13/1
  [eth_eof] -> Logical13/1
  Logical13/1 -> Counter14/2
  [hdr_send_end] -> Logical13/2
  [eth_eof] -> Logical14/1
  Logical14/1 -> Counter15/2
  [interpacket_end] -> Logical14/2
  Relational2/1 -> posedge1/1(in)
  [eth_reset] -> Counter14/1
  posedge14/1(out) -> Logical11/1, [interpacket_end]
  [eth_reset] -> Counter15/1
  Counter15/1 -> Slice14/1
  FIFO/3 -> [queue_perc_full]
  Slice13/1 -> Logical12/2
  Slice14/1 -> [interpacket_valid], Counter13/2
  tgbe0/4(tx_afull) -> Delay30/1
  Delay94/1 -> tgbe0/6(tx_end_of_frame)
  queue_perc_full/1(sim_out) -> Terminator21/1
  [queue_perc_full] -> Delay124/1
  Delay124/1 -> queue_perc_full/1(out_reg)
  queue_empty/1(sim_out) -> Terminator24/1
  [queue_empty] -> Delay125/1
  Delay125/1 -> queue_empty/1(out_reg)
  eth_packet_length_cnt/1(sim_out) -> Terminator25/1
  [packet_length_cnt] -> Delay126/1
  Delay126/1 -> eth_packet_length_cnt/1(out_reg)
  eth_interpacket_length_cnt/1(sim_out) -> Terminator26/1
  [interpacket_length_cnt] -> Delay127/1
  Delay127/1 -> eth_interpacket_length_cnt/1(out_reg)
  Logical15/1 -> Delay68/1
  Slice/1 -> Logical15/1
  [stokes_sync_out] -> Delay51/1
  Delay51/1 -> Logical15/2
  Counter6/1 -> Delay74/1
  [packetiser_of] -> Delay57/1
  posedge15/1(out) -> Counter6/2
  Delay57/1 -> posedge15/1(in)
  [eth_reset] -> Delay58/1
  Delay58/1 -> Counter6/1
  Delay59/1 -> [vacc_1], Reinterpret/1
  Delay83/1 -> Logical2/1
  Delay105/1 -> Reinterpret7/1
  Delay106/1 -> Logical2/2
  Delay128/1 -> Reinterpret1/1
  Delay129/1 -> Logical2/3
  Delay130/1 -> Reinterpret2/1
  Delay131/1 -> Logical2/4
  Delay132/1 -> Reinterpret3/1
  Delay133/1 -> Logical4/1
  Delay134/1 -> Reinterpret4/1
  Delay135/1 -> Logical4/2
  Delay136/1 -> Reinterpret5/1
  Delay137/1 -> Logical4/3
  Delay138/1 -> Reinterpret6/1
  Delay139/1 -> Logical4/4
  packetizer/5(perc_full) -> [packetiser_perc_full]
  Delay52/1 -> packetizer/3(reset)
  [eth_reset] -> Delay52/1
  packetizer/6(done) -> [packetiser_done]
  Reinterpret/1 -> Concat2/1
  Reinterpret1/1 -> Concat2/3
  Reinterpret2/1 -> Concat2/4
  Reinterpret3/1 -> Concat1/1
  Reinterpret4/1 -> Concat1/2
  Reinterpret5/1 -> Concat1/3
  Reinterpret6/1 -> Concat1/4
  Reinterpret7/1 -> Concat2/2
  Counter16/1 -> [hdr_length_cnt], Relational5/1
  Logical18/1 -> Counter16/1
  hdr_size/1 -> Relational5/2
  Relational5/1 -> posedge8/1(in)
  [eth_reset] -> Logical18/2
  [interpacket_end] -> Logical19/1
  Logical19/1 -> Counter17/2
  [hdr_send_end] -> Logical19/2
  posedge8/1(out) -> Logical18/1, [hdr_send_end]
  [eth_reset] -> Counter17/1
  Counter17/1 -> Slice8/1
  Slice8/1 -> Logical17/1, Counter16/2
  magic_no/1 -> Concat4/1
  Concat6/1 -> Concat4/5
  [eth_reset] -> Delay144/1
  sub_frame_cnt/1 -> Relational6/1, [hdr_subframe_cnt], Concat4/3
  Logical21/1 -> sub_frame_cnt/1
  Delay144/1 -> Logical21/2
  [eth_eof] -> sub_frame_cnt/2
  Concat4/1 -> [hdr_dout]
  posedge11/1(out) -> Logical9/1
  Delay141/1 -> Mux/2
  [hdr_dout] -> Slice10/1, Slice9/1
  Delay140/1 -> Mux/3
  Slice9/1 -> Delay141/1
  Slice10/1 -> Delay140/1
  [queue_dout] -> Delay3/1
  Concat5/1 -> [eth_mux_select], Delay142/1
  [eth_hdr_tx_valid] -> Logical22/1, Inverter3/1
  Relational6/1 -> Logical21/1
  [eth_reset] -> Inverter1/1
  Inverter1/1 -> Logical17/2
  Logical17/1 -> [eth_hdr_tx_valid]
  Delay142/1 -> Mux/1
  Inverter3/1 -> Concat5/1
  [hdr_length_cnt] -> Slice11/1
  Logical22/1 -> Concat5/2
  Slice11/1 -> Logical22/2
  Delay160/1 -> Delay27/1
  Delay161/1 -> Delay26/1
  Delay162/1 -> Delay25/1
  Delay163/1 -> Delay24/1
  Delay164/1 -> Delay23/1
  Delay165/1 -> Delay22/1
  Delay166/1 -> Delay21/1
  Delay167/1 -> Delay20/1
  Inverter2/1 -> Logical12/1
  [eth_hdr_tx_valid] -> Logical20/2
  Delay49/1 -> tgbe0/3(tx_valid)
  [eth_data_tx_valid] -> Logical20/1
  Delay3/1 -> Mux/4
  Delay5/1 -> Slice17/1
  eth_interframe_length_1/1 -> eth_packets_per_accum_window/1(sim_1)
  eth_packets_per_accum_window/1(in_reg) -> Delay5/1
  "1 "/1 -> AddSub/2
  Slice16/1 -> Relational4/2
  [eth_packets_per_accum_window] -> Delay170/1
  Slice17/1 -> [eth_packets_per_accum_window]
  Delay170/1 -> Concat4/4
  Shift/1 -> AddSub/1
  Delay171/1 -> Slice19/1
  eth_interframe_length_2/1 -> eth_data_size_per_packet/1(sim_1)
  eth_data_size_per_packet/1(in_reg) -> Delay171/1
  Slice19/1 -> [eth_data_size_per_packet]
  posedge/1(out) -> Delay151/1
  eth_cycles_per_packet/1(sim_out) -> Terminator16/1
  Delay50/1 -> eth_cycles_per_packet/1(out_reg)
  AddSub/1 -> Delay48/1
  Delay27/1 -> simple_bram_vacc_i_even/2(din)
  sync_next_pps/1(in_reg) -> Slice18/1
  Signal Builder1/1(Signal 1) -> sync_next_pps/1(sim_1)
  posedge16/1(out) -> Delay168/1
  Slice18/1 -> posedge16/1(in)
  Delay168/1 -> [sync_next_pps], Counter18/2
  Logical16/1 -> [sync_pulse]
  [sync_pulse] -> Delay56/1
  Counter18/1 -> Slice15/1
  Logical/1 -> posedge9/1(in)
  Delay172/1 -> Counter18/1
  roach_led0/1 -> Terminator27/1
  roach_led1/1 -> Terminator31/1
  roach_led2/1 -> Terminator32/1
  roach_led3/1 -> Terminator33/1
  roach_led4/1 -> Terminator37/1
  roach_led5/1 -> Terminator34/1
  roach_led6/1 -> Terminator36/1
  roach_led7/1 -> Terminator35/1
  tgbe0/5(tx_overflow) -> [eth_tx_of], Delay11/1
  [eth_data_size_per_packet] -> Shift/1
  Delay48/1 -> Delay50/1, Relational2/2
  Logical23/1 -> Logical16/1
  Delay77/1 -> Logical16/2
  [sync_pulse] -> Delay172/1
  posedge5/1(out) -> Delay77/1
  [pps] -> Logical23/1
  Delay8/1 -> Slice12/1
  Slice12/1 -> [eth_eof_led]
  Slice1/1 -> [acc_trig_led]
  roach_sma_j10/1 -> Terminator38/1
  Delay108/1 -> roach_sma_j10/1
  Logical27/1 -> [noise_diode_on], Delay108/1
  err_clear_sim2/1 -> noise_diode_en/1(sim_1)
  noise_diode_en/1(in_reg) -> Slice4/1
  Slice4/1 -> Delay107/1, [noise_diode_enable]
  Counter20/1 -> [noise_diode_on_cnt], Relational8/1
  Logical28/1 -> Counter20/1
  Delay111/1 -> Relational8/2
  Relational8/1 -> posedge6/1(in)
  [noise_diode_on_end] -> Logical29/1
  Logical29/1 -> Counter21/2
  [noise_diode_off_end] -> Logical29/2
  posedge6/1(out) -> Logical28/1, [noise_diode_on_end]
  Logical33/1 -> Counter21/1, Logical28/2
  Counter21/1 -> Slice23/1
  Slice23/1 -> Logical31/1, Inverter5/1, [noise_diode_duty_cycle_on]
  err_clear_sim5/1 -> noise_diode_on_length/1(sim_1)
  noise_diode_on_length/1(in_reg) -> Delay111/1
  Counter4/1 -> [noise_diode_off_cnt], Relational7/1
  Logical25/1 -> Counter4/1
  Delay109/1 -> Relational7/2
  Relational7/1 -> posedge4/1(in)
  [eth_reset] -> Logical25/2
  [noise_diode_on_end] -> Logical26/1
  Logical26/1 -> Counter5/2
  [noise_diode_off_end] -> Logical26/2
  posedge4/1(out) -> Logical25/1, [noise_diode_off_end]
  [eth_reset] -> Counter5/1
  Counter5/1 -> Slice22/1
  Slice22/1 -> Logical30/1, [noise_diode_duty_cycle_off]
  err_clear_sim6/1 -> noise_diode_off_length/1(sim_1)
  noise_diode_off_length/1(in_reg) -> Delay109/1
  [noise_diode_duty_cycle_on] -> Delay146/1
  Logical30/1 -> Counter4/2
  [acc_trig] -> Logical30/2
  Logical31/1 -> Counter20/2
  [acc_trig] -> Delay123/1
  Logical32/1 -> Logical29/3
  Inverter5/1 -> Logical32/4
  [noise_diode_enable] -> Logical32/2
  [noise_diode_enable] -> posedge17/1(in)
  posedge17/1(out) -> Logical33/1
  [eth_reset] -> Logical33/2
  [stokes_enable] -> Delay245/1
  [noise_diode_on] -> Concat6/1
  acc_trig_/1 -> Scope/2
  Delay115/1 -> acc_trig_/1
  noise_diode_on_end_/1 -> Scope/3
  Delay117/1 -> noise_diode_on_end_/1
  noise_diode_duty_cycle_on_/1 -> Scope/4
  Delay118/1 -> noise_diode_duty_cycle_on_/1
  [acc_trig] -> Delay115/1
  [noise_diode_duty_cycle_on] -> Delay118/1
  [noise_diode_on_end] -> Delay117/1
  hdr_size2/1 -> Delay120/1, Delay121/1
  roach_gpio_a_enable_not/1 -> Terminator39/1
  roach_gpio_b_enable_not/1 -> Terminator40/1
  Delay120/1 -> roach_gpio_a_enable_not/1
  Delay121/1 -> roach_gpio_b_enable_not/1
  noise_diode_on_cnt_/1 -> Scope/6
  Delay122/1 -> noise_diode_on_cnt_/1
  [noise_diode_on_cnt] -> Delay122/1
  Delay123/1 -> Logical32/1
  err_clear_sim7/1 -> noise_diode_duty_cycle_en/1(sim_1)
  noise_diode_duty_cycle_en/1(in_reg) -> Slice24/1
  Slice24/1 -> Inverter6/1
  Inverter6/1 -> Delay145/1
  Logical34/1 -> Logical27/2
  Delay107/1 -> Logical27/1
  Delay145/1 -> Logical34/1
  Delay146/1 -> Logical34/2
  Delay147/1 -> Counter2/2
  Delay110/1 -> noise_diode_off_end_/1
  [noise_diode_off_end] -> Delay110/1
  eth_reset_/1 -> Scope/1
  Delay119/1 -> eth_reset_/1
  [eth_reset] -> Delay119/1
  noise_diode_off_end_/1 -> Scope/5
  noise_diode_off_cnt_/1 -> Scope/7
  Delay7/1 -> noise_diode_off_cnt_/1
  [noise_diode_off_cnt] -> Delay7/1
  [noise_diode_duty_cycle_off] -> Inverter7/1
  Inverter7/1 -> Logical32/3
  fft_wideband_real/6(of) -> Delay2/1
  fft_overflow_cnt/1(sim_out) -> Terminator22/1
  Counter19/1 -> Delay4/1
  Delay4/1 -> fft_overflow_cnt/1(out_reg)
  Delay2/1 -> Slice3/1, [fft_overflow]
  [pfb_sync_out] -> Counter19/1
  Slice3/1 -> Counter19/2
  fft_wideband_real/2(out00) -> Delay79/1
  fft_wideband_real/4(out10) -> Delay81/1
  c_to_ri/1 -> Delay95/1
  c_to_ri/2 -> Delay96/1
  c_to_ri1/1 -> Delay97/1
  c_to_ri1/2 -> Delay98/1
  fft_wideband_real/3(out01) -> Delay80/1
  fft_wideband_real/5(out11) -> Delay82/1
  c_to_ri2/1 -> Delay99/1
  c_to_ri2/2 -> Delay100/1
  c_to_ri3/1 -> Delay101/1
  c_to_ri3/2 -> Delay102/1
  [fft_sync_out] -> stokes_odd/1(sync_in)
  Delay1/1 -> Delay103/1
  Delay79/1 -> c_to_ri/1
  Delay80/1 -> c_to_ri2/1
  Delay81/1 -> c_to_ri1/1
  Delay82/1 -> c_to_ri3/1
  Delay95/1 -> stokes_even/2(left_real)
  Delay96/1 -> stokes_even/3(left_imag)
  Delay97/1 -> stokes_even/4(right_real)
  Delay98/1 -> stokes_even/5(right_imag)
  Delay99/1 -> stokes_odd/2(left_real)
  Delay100/1 -> stokes_odd/3(left_imag)
  Delay101/1 -> stokes_odd/4(right_real)
  Delay102/1 -> stokes_odd/5(right_imag)
  Delay103/1 -> [fft_sync_out], stokes_even/1(sync_in)
  stokes_even/1(sync_out) -> [stokes_sync_out]
  stokes_even/2(stokes_i) -> Terminator42/1
  stokes_even/3(stokes_q) -> [stokes_q_even]
  stokes_even/4(stokes_u) -> [stokes_u_even]
  stokes_even/5(stokes_v) -> Terminator43/1
  stokes_odd/1(sync_out) -> Terminator41/1
  stokes_odd/2(stokes_i) -> Terminator44/1
  fft_wideband_real/1(sync_out) -> Delay1/1
  stokes_even/6(l_power) -> [l_power_even]
  stokes_even/8(r_power) -> [r_power_even]
  stokes_odd/3(stokes_q) -> [stokes_q_odd]
  stokes_odd/5(stokes_v) -> Terminator45/1
  stokes_odd/6(l_power) -> [l_power_odd]
  [acc_trig] -> Logical31/2
  Delay151/1 -> [acc_trig]
  katadc/15(data_valid) -> Terminator14/1
  Counter23/1 -> [clk_frequency_cnt], Register19/1
  Register19/1 -> Relational/1, Relational9/1, clk_frequency/1(out_reg)
  clk_frequency/1(sim_out) -> [clk_frequency_reg]
  [pps] -> Counter23/1, Register19/2
  Constant10/1 -> Relational/2
  Constant37/1 -> Relational9/2
  Relational/1 -> Logical7/1
  Relational9/1 -> Logical7/2
  Logical7/1 -> [clk_bad]
  [pps] -> Delay60/1
  Delay60/1 -> Counter/1
  Counter/1 -> Slice5/1
  Slice5/1 -> Delay64/1
  Delay64/1 -> roach_led7/1
  [eth_up] -> Delay6/1
  Delay47/1 -> roach_led6/1
  Delay6/1 -> Delay47/1
  Delay65/1 -> roach_led5/1
  [eth_eof_led] -> Delay63/1
  Delay63/1 -> Delay65/1
  Delay67/1 -> roach_led4/1
  [noise_diode_led] -> Delay61/1
  Delay61/1 -> Delay67/1
  Delay39/1 -> roach_led2/1
  Delay44/1 -> roach_led3/1
  Delay66/1 -> roach_led1/1
  [clk_bad] -> Delay46/1
  Delay46/1 -> Delay66/1
  Delay62/1 -> negedge_delay3/1(in)
  negedge_delay3/1(out) -> Delay152/1
  [of_led] -> Delay62/1
  Delay152/1 -> roach_led0/1
  [sync_pulse] -> Logical35/1, Counter22/1
  Constant11/1 -> time_lsb/1(sim_1)
  Counter22/1 -> [rtc]
  Constant12/1 -> time_msb/1(sim_1)
  Concat8/1 -> Reinterpret8/1
  time_msb/1(in_reg) -> Concat8/1
  time_lsb/1(in_reg) -> Concat8/2
  Counter24/1 -> Relational10/1
  window_size1/1 -> Relational10/2
  Relational10/1 -> posedge18/1(in)
  posedge18/1(out) -> Logical38/1, Logical35/2, [usec_tick]
  Counter25/1 -> [dsp_delay_cnt], Register1/1
  Register1/1 -> Delay153/1
  [sync_pulse] -> Counter25/1
  [acc_trig] -> Logical37/1
  [wait_for_pps] -> Counter26/1
  [acc_trig] -> Logical36/1
  Logical36/1 -> Counter26/2
  Logical37/1 -> Register1/2
  Delay143/1 -> Logical37/2
  [usec_tick] -> Counter25/2
  [rtc] -> Register2/1
  Register2/1 -> Delay154/1
  [acc_trig] -> Register2/2
  dsp_delay/1(sim_out) -> Terminator15/1
  Delay153/1 -> Delay155/1, [dsp_delay]
  Delay155/1 -> dsp_delay/1(out_reg)
  last_timestamp_lsb/1(sim_out) -> Terminator47/1
  Delay156/1 -> last_timestamp_lsb/1(out_reg)
  [dsp_delay] -> AddSub1/2
  Delay154/1 -> AddSub1/1
  last_timestamp_msb/1(sim_out) -> Terminator48/1
  Delay157/1 -> last_timestamp_msb/1(out_reg)
  AddSub1/1 -> Slice27/1, Slice26/1, [timestamp]
  Slice26/1 -> Delay157/1
  Slice27/1 -> Delay156/1
  [timestamp] -> Reinterpret9/1
  Slice15/1 -> [wait_for_pps], Logical23/2
  Reinterpret8/1 -> Counter22/2
  Counter26/1 -> Slice28/1
  Slice28/1 -> Logical36/2, Delay143/1
  Reinterpret9/1 -> Concat4/2
  acc_trig__/1 -> Scope2/2
  Delay158/1 -> acc_trig__/1
  [acc_trig] -> Delay158/1
  sync_pulse_/1 -> Scope2/1
  Delay173/1 -> sync_pulse_/1
  [sync_pulse] -> Delay173/1
  timestamp_/1 -> Scope2/6
  Delay169/1 -> timestamp_/1
  [timestamp] -> Delay169/1
  Delay174/1 -> rtc_/1
  [rtc] -> Delay174/1
  rtc_/1 -> Scope2/5
  dsp_delay_/1 -> Scope2/4
  Delay159/1 -> dsp_delay_/1
  [dsp_delay] -> Delay159/1
  dsp_delay_cnt_/1 -> Scope2/3
  Delay175/1 -> dsp_delay_cnt_/1
  [dsp_delay_cnt] -> Delay175/1
  usec_tick_/1 -> Scope2/7
  Delay176/1 -> usec_tick_/1
  [usec_tick] -> Delay176/1
  [wait_for_pps] -> Logical38/2
  Logical38/1 -> Counter24/1
  Delay177/1 -> [eth_reset]
  wait_for_pps_/1 -> Scope2/8
  Delay178/1 -> wait_for_pps_/1
  [wait_for_pps] -> Delay178/1
  another1/1 -> AddSub2/2
  [eth_packets_per_accum_window] -> Delay206/1
  AddSub2/1 -> Delay200/1
  Logical35/1 -> Counter22/3
  Delay179/1 -> Delay199/1
  Delay180/1 -> Delay254/1
  Delay181/1 -> Delay255/1
  Delay182/1 -> Delay256/1
  Delay183/1 -> [adc0_or]
  Delay184/1 -> Delay257/1
  Delay185/1 -> Delay258/1
  Delay186/1 -> Delay259/1
  Delay187/1 -> Delay260/1
  Delay188/1 -> [adc1_or]
  Delay189/1 -> Logical/1
  Delay190/1 -> Logical/2
  Delay191/1 -> Logical/3
  Delay192/1 -> Logical/4
  Delay193/1 -> katadc/8(atten1)
  Delay194/1 -> katadc/7(en1)
  Delay195/1 -> katadc/6(atten0)
  Delay196/1 -> katadc/5(en0)
  Delay197/1 -> [pps]
  Delay200/1 -> Relational6/2
  [clk_frequency_reg] -> Scope3/2
  pps_/1 -> Scope3/1
  Delay204/1 -> pps_/1
  [pps] -> Delay204/1
  clk_frequency_cnt_/1 -> Scope3/3
  Delay202/1 -> clk_frequency_cnt_/1
  [clk_frequency_cnt] -> Delay202/1
  pps_cnt/1(sim_out) -> Terminator23/1
  Counter7/1 -> Delay76/1
  Delay76/1 -> pps_cnt/1(out_reg)
  Delay87/1 -> Counter7/2
  [sync_pulse] -> Counter7/1
  [pps] -> Delay87/1
  posedge9/1(out) -> Delay197/1
  Mux1/1 -> Delay201/1
  Delay201/1 -> [noise_diode_led]
  [noise_diode_enable] -> Delay213/1
  [noise_diode_on] -> Delay212/1
  Delay213/1 -> Concat9/1
  Delay212/1 -> Concat9/2
  Concat9/1 -> Delay214/1
  Delay214/1 -> Mux1/1
  Constant15/1 -> Delay215/1
  Constant16/1 -> Delay217/1
  Counter30/1 -> Slice33/1
  Relational11/1 -> posedge19/1(in)
  Counter31/1 -> Relational11/1
  Constant17/1 -> Relational11/2
  Delay203/1 -> Counter31/1, Counter30/1
  posedge19/1(out) -> Delay203/1
  [usec_tick] -> Delay205/1
  Delay205/1 -> Counter31/2
  Slice33/1 -> Delay216/1
  Delay215/1 -> Mux1/2, Mux1/3
  Delay217/1 -> Mux1/5
  Delay216/1 -> Mux1/4
  Delay206/1 -> AddSub2/1
  [fft_overflow] -> Delay42/1
  [packetiser_of] -> Delay9/1
  Delay9/1 -> overflows/3(out_packetiser_of), Logical24/3
  [queue_full] -> Delay43/1
  Delay43/1 -> overflows/4(out_fifo_full), Logical24/4
  [eth_tx_of] -> Delay45/1
  Delay45/1 -> overflows/5(out_eth_tx_of), Logical24/5
  Delay42/1 -> Slice20/1, Slice21/1
  [adc0_or] -> Delay148/1
  Delay148/1 -> overflows/7(out_adc0_or), Logical24/6
  [adc1_or] -> Delay149/1
  Delay149/1 -> overflows/6(out_adc1_or), Logical24/7
  Slice20/1 -> overflows/1(out_fft1_of), Logical24/1
  Logical24/1 -> [of_led]
  overflows/1(sim_out) -> Terminator13/1
  Slice21/1 -> overflows/2(out_fft0_of), Logical24/2
  Delay207/1 -> Delay160/1
  Delay209/1 -> Delay161/1
  Mux7/1 -> Delay162/1
  Mux6/1 -> Delay163/1
  Delay221/1 -> Delay164/1
  Delay223/1 -> Delay165/1
  Mux3/1 -> Delay166/1
  Mux9/1 -> Delay167/1
  stokes_enable/1(in_reg) -> Slice29/1
  accumlation_count1/1 -> stokes_enable/1(sim_1)
  Slice29/1 -> Delay236/1
  Delay236/1 -> [stokes_enable], Delay239/1, Delay240/1, Delay243/1, Delay244/1
  Delay239/1 -> Mux7/1
  Delay240/1 -> Mux6/1
  Delay243/1 -> Mux3/1
  Delay244/1 -> Mux9/1
  Delay245/1 -> Concat6/3
  another2/1 -> Concat6/2
  [stokes_u_odd] -> Delay226/1
  Delay226/1 -> Mux9/3
  [r_phase_odd] -> Delay227/1
  Delay227/1 -> Mux9/2
  [stokes_q_odd] -> Delay224/1
  Delay224/1 -> Mux3/3
  [l_phase_odd] -> Delay225/1
  Delay225/1 -> Mux3/2
  [r_power_odd] -> Delay222/1
  Delay222/1 -> Delay223/1
  [stokes_u_even] -> Delay218/1
  Delay218/1 -> Mux6/3
  [r_phase_even] -> Delay219/1
  Delay219/1 -> Mux6/2
  [stokes_q_even] -> Delay210/1
  Delay210/1 -> Mux7/3
  [l_phase_even] -> Delay211/1
  Delay211/1 -> Mux7/2
  [r_power_even] -> Delay208/1
  Delay208/1 -> Delay209/1
  [l_power_even] -> Delay150/1
  Delay150/1 -> Delay207/1
  [l_power_odd] -> Delay220/1
  Delay220/1 -> Delay221/1
  stokes_even/7(l_phase) -> [l_phase_even]
  stokes_even/9(r_phase) -> [r_phase_even]
  stokes_odd/4(stokes_u) -> [stokes_u_odd]
  stokes_odd/8(r_power) -> [r_power_odd]
  stokes_odd/9(r_phase) -> [r_phase_odd]
  stokes_odd/7(l_phase) -> [l_phase_odd]
  sampling_frequency_mhz/1(sim_out) -> Terminator46/1
  Constant14/1 -> Delay228/1
  Delay228/1 -> sampling_frequency_mhz/1(out_reg)
  coarse_fft_size_nsamp/1(sim_out) -> Terminator49/1
  Constant18/1 -> Delay241/1
  Delay241/1 -> coarse_fft_size_nsamp/1(out_reg)
  fine_fft_size_nsamp/1(sim_out) -> Terminator50/1
  Constant19/1 -> Delay242/1
  Delay242/1 -> fine_fft_size_nsamp/1(out_reg)
  coarse_channel_select/1(sim_out) -> Terminator51/1
  Constant7/1 -> Delay229/1
  Delay229/1 -> coarse_channel_select/1(out_reg)
  accum_samples_per_clk/1(sim_out) -> Terminator54/1
  Constant13/1 -> Delay232/1
  Delay232/1 -> accum_samples_per_clk/1(out_reg)
  Constant1/1 -> adc0_en/1(sim_1)
  Constant3/1 -> adc0_atten/1(sim_1)
  adc1_en/1(in_reg) -> Slice34/1
  adc0_en/1(in_reg) -> Slice31/1
  adc0_atten/1(in_reg) -> Slice32/1
  adc1_atten/1(in_reg) -> Slice30/1
  Slice30/1 -> Delay193/1
  Slice31/1 -> Delay196/1
  Slice32/1 -> Delay195/1
  Slice34/1 -> Delay194/1
  Constant2/1 -> adc1_en/1(sim_1)
  Constant4/1 -> adc1_atten/1(sim_1)
  Mux2/1 -> Delay85/1
  Delay85/1 -> fft_wideband_real/3(in00)
  pfb_fir_real/2(pol1_out1) -> Delay86/1
  Mux4/1 -> Delay88/1
  Delay88/1 -> fft_wideband_real/4(in01)
  pfb_fir_real/3(pol1_out2) -> Delay89/1
  Delay90/1 -> Delay84/1
  Mux5/1 -> Delay91/1
  Delay91/1 -> fft_wideband_real/5(in02)
  pfb_fir_real/4(pol1_out3) -> Delay92/1
  Mux8/1 -> Delay93/1
  pfb_fir_real/5(pol1_out4) -> Delay230/1
  Delay93/1 -> fft_wideband_real/6(in03)
  Mux10/1 -> Delay233/1
  pfb_fir_real/6(pol2_out1) -> Delay231/1
  Delay233/1 -> fft_wideband_real/7(in10)
  Mux11/1 -> Delay235/1
  Delay235/1 -> fft_wideband_real/8(in11)
  pfb_fir_real/7(pol2_out2) -> Delay234/1
  Mux12/1 -> Delay238/1
  pfb_fir_real/8(pol2_out3) -> Delay237/1
  Mux13/1 -> Delay247/1
  pfb_fir_real/9(pol2_out4) -> Delay246/1
  Delay247/1 -> fft_wideband_real/10(in13)
  Delay238/1 -> fft_wideband_real/9(in12)
  Delay86/1 -> Mux2/2
  convert_of/1(dout) -> Mux2/3
  Delay89/1 -> Mux4/2
  convert_of1/1(dout) -> Mux4/3
  Delay92/1 -> Mux5/2
  convert_of2/1(dout) -> Mux5/3
  Delay230/1 -> Mux8/2
  convert_of3/1(dout) -> Mux8/3
  Delay231/1 -> Mux10/2
  convert_of4/1(dout) -> Mux10/3
  Delay234/1 -> Mux11/2
  convert_of5/1(dout) -> Mux11/3
  convert_of6/1(dout) -> Mux12/3
  Delay237/1 -> Mux12/2
  Delay246/1 -> Mux13/2
  convert_of7/1(dout) -> Mux13/3
  bypass_pfb/1(in_reg) -> Delay248/1
  Constant20/1 -> bypass_pfb/1(sim_1)
  Delay248/1 -> Slice35/1
  Slice35/1 -> [bypass_pfb]
  [bypass_pfb] -> Mux2/1
  [bypass_pfb] -> Mux4/1
  [bypass_pfb] -> Mux5/1
  [bypass_pfb] -> Mux8/1
  [bypass_pfb] -> Mux10/1
  [bypass_pfb] -> Mux11/1
  [bypass_pfb] -> Mux12/1
  [bypass_pfb] -> Mux13/1
  Delay199/1 -> [adc_data0_0]
  Delay254/1 -> [adc_data0_1]
  Delay255/1 -> [adc_data0_2]
  Delay256/1 -> [adc_data0_3]
  Delay257/1 -> [adc_data1_0]
  Delay258/1 -> [adc_data1_1]
  Delay259/1 -> [adc_data1_2]
  Delay260/1 -> [adc_data1_3]
  [adc_data0_0] -> Delay54/1
  [adc_data0_1] -> Delay55/1
  [adc_data0_2] -> Delay198/1
  [adc_data0_3] -> Delay249/1
  [adc_data1_0] -> Delay250/1
  [adc_data1_1] -> Delay251/1
  [adc_data1_2] -> Delay252/1
  [adc_data1_3] -> Delay253/1
  [adc_data0_0] -> convert_of/1(din)
  [adc_data0_1] -> convert_of1/1(din)
  [adc_data0_2] -> convert_of2/1(din)
  [adc_data0_3] -> convert_of3/1(din)
  [adc_data1_3] -> convert_of7/1(din)
  [adc_data1_2] -> convert_of6/1(din)
  [adc_data1_1] -> convert_of5/1(din)
  [adc_data1_0] -> convert_of4/1(din)
  [adc_data0_0] -> Delay262/1
  Delay262/1 -> Reinterpret10/1
  Delay269/1 -> Mult3/2, Mult3/1
  Mult3/1 -> Reinterpret12/1
  Delay270/1 -> Accumulator2/1
  Accumulator2/1 -> Delay271/1
  Relational12/1 -> Delay292/1
  Relational13/1 -> Delay290/1
  Register3/1 -> Delay283/1, Relational12/1, Relational13/1
  Counter27/1 -> Relational14/1
  Relational14/1 -> posedge3/1(in)
  posedge3/1(out) -> Counter27/1, Delay275/1
  adc_threshold_acc_length/1(in_reg) -> Delay274/1
  upper_adc_threshold/1(in_reg) -> Delay272/1
  lower_adc_threshold/1(in_reg) -> Delay273/1
  Delay272/1 -> [adc_upper_threshold]
  Delay273/1 -> [adc_lower_threshold]
  Delay274/1 -> Relational14/2
  Delay275/1 -> [adc_threshold_acc_trig]
  [adc_lower_threshold] -> Relational13/2
  [adc_upper_threshold] -> Relational12/2
  [adc_data1_0] -> Delay266/1
  Delay266/1 -> Reinterpret11/1
  Delay280/1 -> Mult1/1, Mult1/2
  Mult1/1 -> Reinterpret13/1
  Delay281/1 -> Accumulator1/1
  Accumulator1/1 -> Delay282/1
  Relational15/1 -> Delay288/1
  Relational16/1 -> Delay286/1
  [adc_lower_threshold] -> Relational16/2
  [adc_upper_threshold] -> Relational15/2
  Delay283/1 -> adc0_threshold_acc/1(out_reg)
  Register6/1 -> Relational15/1, Delay284/1, Relational16/1
  Delay284/1 -> adc1_threshold_acc/1(out_reg)
  Delay292/1 -> Logical39/1
  Delay288/1 -> Logical39/2
  Delay290/1 -> Logical40/1
  Delay286/1 -> Logical40/2
  Logical39/1 -> Delay295/1
  Logical40/1 -> Delay296/1
  Delay294/1 -> [adc_over_threshold], adc_over_threshold/1(out_reg)
  Delay293/1 -> [adc_under_threshold], adc_under_threshold/1(out_reg)
  Delay295/1 -> negedge_delay2/1(in)
  Delay296/1 -> negedge_delay1/1(in)
  negedge_delay1/1(out) -> Slice36/1
  negedge_delay2/1(out) -> Slice25/1
  [adc_over_threshold] -> Delay297/1
  Delay297/1 -> Delay39/1
  [adc_under_threshold] -> Delay298/1
  Delay298/1 -> Delay44/1
  Reinterpret10/1 -> Delay269/1
  Reinterpret11/1 -> Delay280/1
  Slice25/1 -> Delay294/1
  Slice36/1 -> Delay293/1
  Delay285/1 -> Register6/2
  Delay282/1 -> Register6/1
  Delay261/1 -> Register3/2
  Delay271/1 -> Register3/1
  Reinterpret12/1 -> Delay270/1
  Reinterpret13/1 -> Delay281/1
  [adc_threshold_acc_trig] -> Delay261/1, Accumulator2/2
  [adc_threshold_acc_trig] -> Delay285/1, Accumulator1/2
